simulink model "MPCtest1_real_44_180"  (Simulink 8.7)
settings: Solver=VariableStepAuto  StartTime=0.0  StopTime=16  RelTol=1e-3
libraries: neural x44, simulink x4, Solver_SF x1
(part 1 of 3)
settings Model: Creator=zch  LastModifiedBy=zch
settings DataIOCC: LimitDataPoints=off  SaveFormat=Dataset
settings DebuggingCC: UnderspecifiedInitializationDetection=Simplified  MergeDetectMultiDrivingBlocksExec=error
settings HardwareCC: ProdBitPerPointer=64  ProdLargestAtomicFloat=Float  ProdIntDivRoundTo=Zero  ProdEndianess=LittleEndian  ProdWordSize=64  ProdHWDeviceType=Intel->x86-64 (Windows64)
settings ModelReferenceCC: PropagateSignalLabelsOutOfModel=on
settings ConfigComp: CovModelRefEnable=off

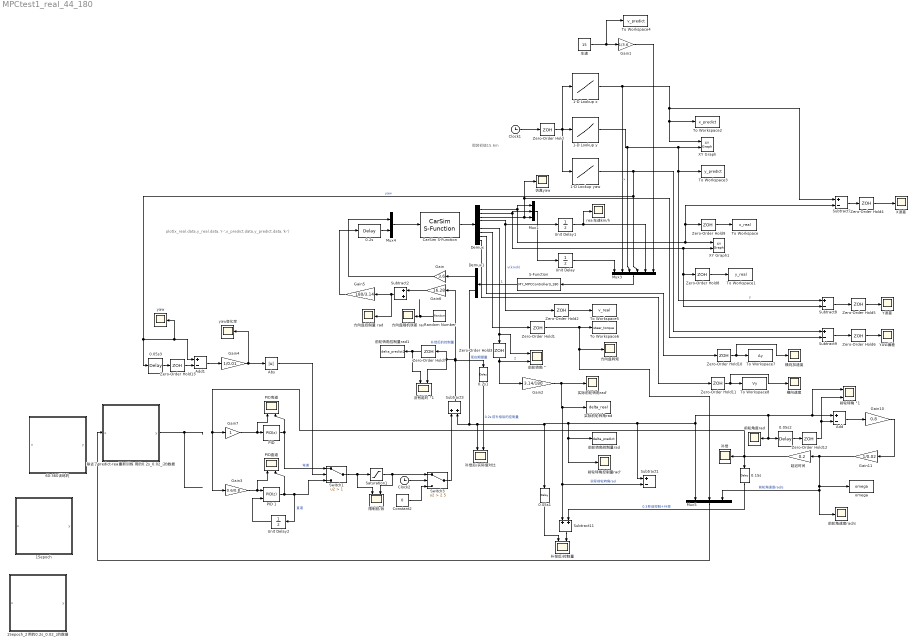
== system MPCtest1_real_44_180 ==
  note: plot(x_real.data,y_real.data,'r-',x_predict.data,y_predict.data,'k-')
  note: 假装初值15.6m
  0.05s1 : TransportDelay  DelayTime=0.05  PadeOrder=2
  0.05s2 : TransportDelay  DelayTime=0.02  PadeOrder=2
  0.05s3 : TransportDelay  DelayTime=0.01  PadeOrder=2
  0.15s : TransportDelay  DelayTime=0.15  PadeOrder=2
  0.2s : TransportDelay  DelayTime=0.2  PadeOrder=2
  0.2s1 : TransportDelay  DelayTime=0.2  PadeOrder=2
  1-D Lookup x : Lookup_n-D  NumberOfTableDimensions=1  BreakpointsForDimension1=|  Table=|  InternalRulePriority=Speed  RndMeth=Simplest  InputSameDT=on
      | [0
      | 0.018
      | 0.036
      | 0.054
      | 0.072
      | 0.09
      | 0.108
      | 0.126
      | 0.144
      | 0.162
      | 0.18
      | 0.198
      | 0.216
      | 0.234
      | 0.252
      | 0.27
      | 0.288
      | 0.306
      | 0.324
      | 0.342
      | 0.36
      | 0.378
      | 0.396
      | 0.414
      | 0.432
      | 0.45
      | 0.468
      | 0.486
      | 0.504
      | 0.522
      | 0.54
      | 0.558
      | 0.576
      | 0.594
      | 0.612
      | 0.63
      | 0.648
      | 0.666
      | 0.684
      | 0.702
      | 0.72
      | 0.738
      | 0.756
      | 0.774
      | 0.792
      | 0.81
      | 0.828
      | 0.846
      | 0.864
      | 0.882
      | 0.9
      | 0.918
      | 0.936
      | 0.954
      | 0.972
      | 0.99
      | 1.008
      | 1.026
      | 1.044
      | 1.062
      | 1.08
      | 1.098
      | 1.116
      | 1.134
      | 1.152
      | 1.17
      | 1.188
      | 1.206
      | 1.224
      | 1.242
      | 1.26
      | 1.278
      | 1.296
      | 1.314
      | 1.332
      | 1.35
      | 1.368
      | 1.386
      | 1.404
      | 1.422
      | 1.44
      | 1.458
      | 1.476
      | 1.494
      | 1.512
      | 1.53
      | 1.548
      | 1.566
      | 1.584
      | 1.602
      | 1.62
      | 1.638
      | 1.656
      | 1.674
      | 1.692
      | 1.71
      | 1.728
      | 1.746
      | 1.764
      | 1.782
      | 1.8
      | 1.818
      | 1.836
      | 1.854
      | 1.872
      | 1.89
      | 1.908
      | 1.926
      | 1.944
      | 1.962
      | 1.98
      | 1.998
      | 2.016
      | 2.034
      | 2.052
      | 2.07
      | 2.088
      | 2.106
      | 2.124
      | 2.142
      | 2.16
      | 2.178
      | 2.196
      | 2.214
      | 2.232
      | 2.25
      | 2.268
      | 2.286
      | 2.304
      | 2.322
      | 2.34
      | 2.358
      | 2.376
      | 2.394
      | 2.412
      | 2.43
      | 2.448
      | 2.466
      | 2.484
      | 2.502
      | 2.52
      | 2.538
      | 2.556
      | 2.574
      | 2.592
      | 2.61
      | 2.628
      | 2.646
      | 2.664
      | 2.682
      | 2.7
      | 2.718
      | 2.736
      | 2.754
      | 2.772
      | 2.79
      | 2.808
      | 2.826
      | 2.844
      | 2.862
      | 2.88
      | 2.898
      | 2.916
      | 2.934
      | 2.952
      | 2.97
      | 2.988
      | 3.006
      | 3.024
      | 3.042
      | 3.06
      | 3.078
      | 3.096
      | 3.114
      | 3.132
      | 3.15
      | 3.168
      | 3.186
      | 3.204
      | 3.222
      | 3.24
      | 3.258
      | 3.276
      | 3.294
      | 3.312
      | 3.33
      | 3.348
      | 3.366
      | 3.384
      | 3.402
      | 3.42
      | 3.438
      | 3.456
      | 3.474
      | 3.492
      | 3.51
      | 3.528
      | 3.546
      | 3.564
      | 3.582
      | 3.6
      | 3.61439994
      | 3.62879988
      | 3.64319982
      | 3.65759976
      | 3.6719997
      | 3.68639964
      | 3.70079958
      | 3.71519952
      | 3.72959946
      | 3.7439994
      | 3.75839934
      | 3.77279928
      | 3.78719922
      | 3.80159916
      | 3.8159991
      | 3.83039904
      | 3.84479898
      | 3.85919892
      | 3.87359886
      | 3.8879988
      | 3.90239874
      | 3.91679868
      | 3.93119862
      | 3.94559856
      | 3.9599985
      | 3.97439844
      | 3.98879838
      | 4.00319832
      | 4.01759826
      | 4.0319982
      | 4.04639814
      | 4.06079808
      | 4.07519802
      | 4.08959796
      | 4.1039979
      | 4.11839784
      | 4.13279778
      | 4.14719772
      | 4.16159766
      | 4.1759976
      | 4.19039754
      | 4.20479748
      | 4.21919742
      | 4.23359736
      | 4.2479973
      | 4.26239724
      | 4.27679718
      | 4.29119712
      | 4.30559706
      | 4.319997
      | 4.33439694
      | 4.34879688
      | 4.36319682
      | 4.37759676
      | 4.3919967
      | 4.40639664
      | 4.42079658
      | 4.43519652
      | 4.44959646
      | 4.4639964
      | 4.47839634
      | 4.49279628
      | 4.50719622
      | 4.52159616
      | 4.5359961
      | 4.55039604
      | 4.56479598
      | 4.57919592
      | 4.59359586
      | 4.6079958
      | 4.62239574
      | 4.63679568
      | 4.65119562
      | 4.66559556
      | 4.6799955
      | 4.69439544
      | 4.70879538
      | 4.72319532
      | 4.73759526
      | 4.7519952
      | 4.76639514
      | 4.78079508
      | 4.79519502
      | 4.80959496
      | 4.8239949
      | 4.83839484
      | 4.85279478
      | 4.86719472
      | 4.88159466
      | 4.8959946
      | 4.91039454
      | 4.92479448
      | 4.93919442
      | 4.95359436
      | 4.9679943
      | 4.98239424
      | 4.99679418
      | 5.01119412
      | 5.02559406
      | 5.039994
      | 5.05439394
      | 5.06879388
      | 5.08319382
      | 5.09759376
      | 5.1119937
      | 5.12639364
      | 5.14079358
      | 5.15519352
      | 5.16959346
      | 5.1839934
      | 5.19839334
      | 5.21279328
      | 5.22719322
      | 5.24159316
      | 5.2559931
      | 5.27039304
      | 5.28479298
      | 5.29919292
      | 5.31359286
      | 5.3279928
      | 5.34239274
      | 5.35679268
      | 5.37119262
      | 5.38559256
      | 5.3999925
      | 5.41439244
      | 5.42879238
      | 5.44319232
      | 5.45759226
      | 5.4719922
      | 5.48639214
      | 5.50079208
      | 5.51519202
      | 5.52959196
      | 5.5439919
      | 5.55839184
      | 5.57279178
      | 5.58719172
      | 5.60159166
      | 5.6159916
      | 5.63039154
      | 5.64479148
      | 5.65919142
      | 5.67359136
      | 5.6879913
      | 5.70239124
      | 5.71679118
      | 5.73119112
      | 5.74559106
      | 5.759991
      | 5.77439094
      | 5.78879088
      | 5.80319082
      | 5.81759076
      | 5.8319907
      | 5.84639064
      | 5.86079058
      | 5.87519052
      | 5.88959046
      | 5.9039904
      | 5.91839034
      | 5.93279028
      | 5.94719022
      | 5.96159016
      | 5.9759901
      | 5.99039004
      | 6.00478998
      | 6.01918992
      | 6.03358986
      | 6.0479898
      | 6.06238974
      | 6.07678968
      | 6.09118962
      | 6.10558956
      | 6.1199895
      | 6.13438944
      | 6.14878938
      | 6.16318932
      | 6.17758926
      | 6.1919892
      | 6.20638914
      | 6.22078908
      | 6.23518902
      | 6.24958896
      | 6.2639889
      | 6.27838884
      | 6.29278878
      | 6.30718872
      | 6.32158866
      | 6.3359886
      | 6.35038854
      | 6.36478848
      | 6.37918842
      | 6.39358836
      | 6.4079883
      | 6.42238824
      | 6.43678818
      | 6.45118812
      | 6.46558806
      | 6.479988
      | 6.49438794
      | 6.50878788
      | 6.52318782
      | 6.53758776
      | 6.5519877
      | 6.56638764
      | 6.58078758
      | 6.59518752
      | 6.60958746
      | 6.6239874
      | 6.63838734
      | 6.65278728
      | 6.66718722
      | 6.68158716
      | 6.6959871
      | 6.71038704
      | 6.72478698
      | 6.73918692
      | 6.75358686
      | 6.7679868
      | 6.78238674
      | 6.79678668
      | 6.81118662
      | 6.82558656
      | 6.8399865
      | 6.85438644
      | 6.86878638
      | 6.88318632
      | 6.89758626
      | 6.9119862
      | 6.92638614
      | 6.94078608
      | 6.95518602
      | 6.96958596
      | 6.9839859
      | 6.99838584
      | 7.01278578
      | 7.02718572
      | 7.04158566
      | 7.0559856
      | 7.07038554
      | 7.08478548
      | 7.09918542
      | 7.11358536
      | 7.1279853
      | 7.14238524
      | 7.15678518
      | 7.17118512
      | 7.18558506
      | 7.199985
      | 7.21438494
      | 7.22878488
      | 7.24318482
      | 7.25758476
      | 7.2719847
      | 7.28638464
      | 7.30078458
      | 7.31518452
      | 7.32958446
      | 7.3439844
      | 7.35838434
      | 7.37278428
      | 7.38718422
      | 7.40158416
      | 7.4159841
      | 7.43038404
      | 7.44478398
      | 7.45918392
      | 7.47358386
      | 7.4879838
      | 7.50238374
      | 7.51678368
      | 7.53118362
      | 7.54558356
      | 7.5599835
      | 7.57438344
      | 7.58878338
      | 7.60318332
      | 7.61758326
      | 7.6319832
      | 7.64638314
      | 7.66078308
      | 7.67518302
      | 7.68958296
      | 7.7039829
      | 7.71838284
      | 7.73278278
      | 7.74718272
      | 7.76158266
      | 7.7759826
      | 7.79038254
      | 7.80478248
      | 7.81918242
      | 7.83358236
      | 7.8479823
      | 7.86238224
      | 7.87678218
      | 7.89118212
      | 7.90558206
      | 7.919982
      | 7.93438194
      | 7.94878188
      | 7.96318182
      | 7.97758176
      | 7.9919817
      | 8.00638164
      | 8.02078158
      | 8.03518152
      | 8.04958146
      | 8.0639814
      | 8.07838134
      | 8.09278128
      | 8.10718122
      | 8.12158116
      | 8.123874581
      | 8.141874581
      | 8.159874581
      | 8.177874581
      | 8.195874581
      | 8.213874581
      | 8.231874581
      | 8.249874581
      | 8.267874581
      | 8.285874581
      | 8.303874581
      | 8.321874581
      | 8.339874581
      | 8.357874581
      | 8.375874581
      | 8.393874581
      | 8.411874581
      | 8.429874581
      | 8.447874581
      | 8.465874581
      | 8.483874581
      | 8.501874581
      | 8.519874581
      | 8.537874581
      | 8.555874581
      | 8.573874581
      | 8.591874581
      | 8.609874581
      | 8.627874581
      | 8.645874581
      | 8.663874581
      | 8.681874581
      | 8.699874581
      | 8.717874581
      | 8.735874581
      | 8.753874581
      | 8.771874581
      | 8.789874581
      | 8.807874581
      | 8.825874581
      | 8.843874581
      | 8.861874581
      | 8.879874581
      | 8.897874581
      | 8.915874581
      | 8.933874581
      | 8.951874581
      | 8.969874581
      | 8.987874581
      | 9.005874581
      | 9.023874581
      | 9.041874581
      | 9.059874581
      | 9.077874581
      | 9.095874581
      | 9.113874581
      | 9.131874581
      | 9.149874581
      | 9.167874581
      | 9.185874581
      | 9.203874581
      | 9.221874581
      | 9.239874581
      | 9.257874581
      | 9.275874581
      | 9.293874581
      | 9.311874581
      | 9.329874581
      | 9.347874581
      | 9.365874581
      | 9.383874581
      | 9.401874581
      | 9.419874581
      | 9.437874581
      | 9.455874581
      | 9.473874581
      | 9.491874581
      | 9.509874581
      | 9.527874581
      | 9.545874581
      | 9.563874581
      | 9.581874581
      | 9.599874581
      | 9.617874581
      | 9.635874581
      | 9.653874581
      | 9.671874581
      | 9.689874581
      | 9.707874581
      | 9.725874581
      | 9.743874581
      | 9.761874581
      | 9.779874581
      | 9.797874581
      | 9.815874581
      | 9.833874581
      | 9.851874581
      | 9.869874581
      | 9.887874581
      | 9.905874581
      | 9.923874581
      | 9.941874581
      | 9.959874581
      | 9.977874581
      | 9.995874581
      | 10.01387458
      | 10.03187458
      | 10.04987458
      | 10.06787458
      | 10.08587458
      | 10.10387458
      | 10.12187458
      | 10.13987458
      | 10.15787458
      | 10.17587458
      | 10.19387458
      | 10.21187458
      | 10.22987458
      | 10.24787458
      | 10.26587458
      | 10.28387458
      | 10.30187458
      | 10.31987458
      | 10.33787458
      | 10.35587458
      | 10.37387458
      | 10.39187458
      | 10.40987458
      | 10.42787458
      | 10.44587458
      | 10.46387458
      | 10.48187458
      | 10.49987458
      | 10.51787458
      | 10.53587458
      | 10.55387458
      | 10.57187458
      | 10.58987458
      | 10.60787458
      | 10.62587458
      | 10.64387458
      | 10.66187458
      | 10.67987458
      | 10.69787458
      | 10.71587458
      | 10.73387458
      | 10.75187458
      | 10.76987458
      | 10.78787458
      | 10.80587458
      | 10.82387458
      | 10.84187458
      | 10.85987458
      | 10.87787458
      | 10.89587458
      | 10.91387458
      | 10.93187458
      | 10.94987458
      | 10.96787458
      | 10.98587458
      | 11.00387458
      | 11.02187458
      | 11.03987458
      | 11.05787458
      | 11.07587458
      | 11.09387458
      | 11.11187458
      | 11.12987458
      | 11.14787458
      | 11.16587458
      | 11.18387458
      | 11.20187458
      | 11.21987458
      | 11.23787458
      | 11.25587458
      | 11.27387458
      | 11.29187458
      | 11.30987458
      | 11.32787458
      | 11.34587458
      | 11.36387458
      | 11.38187458
      | 11.39987458
      | 11.41787458
      | 11.43587458
      | 11.45387458
      | 11.47187458
      | 11.48987458
      | 11.50787458
      | 11.52587458
      | 11.54387458
      | 11.56187458
      | 11.57987458
      | 11.59787458
      | 11.61587458
      | 11.63387458
      | 11.65187458
      | 11.66987458
      | 11.68787458
      | 11.70587458
      | 11.72387458
      | ]*4/3
      | [0
      | 0.1
      | 0.2
      | 0.3
      | 0.4
      | 0.5
      | 0.6
      | 0.7
      | 0.8
      | 0.9
      | 1
      | 1.1
      | 1.2
      | 1.3
      | 1.4
      | 1.5
      | 1.6
      | 1.7
      | 1.8
      | 1.9
      | 2
      | 2.1
      | 2.2
      | 2.3
      | 2.4
      | 2.5
      | 2.6
      | 2.7
      | 2.8
      | 2.9
      | 3
      | 3.1
      | 3.2
      | 3.3
      | 3.4
      | 3.5
      | 3.6
      | 3.7
      | 3.8
      | 3.9
      | 4
      | 4.1
      | 4.2
      | 4.3
      | 4.4
      | 4.5
      | 4.6
      | 4.7
      | 4.8
      | 4.9
      | 5
      | 5.1
      | 5.2
      | 5.3
      | 5.4
      | 5.5
      | 5.6
      | 5.7
      | 5.8
      | 5.9
      | 6
      | 6.1
      | 6.2
      | 6.3
      | 6.4
      | 6.5
      | 6.6
      | 6.7
      | 6.8
      | 6.9
      | 7
      | 7.1
      | 7.2
      | 7.3
      | 7.4
      | 7.5
      | 7.6
      | 7.7
      | 7.8
      | 7.9
      | 8
      | 8.1
      | 8.2
      | 8.3
      | 8.4
      | 8.5
      | 8.6
      | 8.7
      | 8.8
      | 8.9
      | 9
      | 9.1
      | 9.2
      | 9.3
      | 9.4
      | 9.5
      | 9.6
      | 9.7
      | 9.8
      | 9.9
      | 10
      | 10.1
      | 10.2
      | 10.3
      | 10.4
      | 10.5
      | 10.6
      | 10.7
      | 10.8
      | 10.9
      | 11
      | 11.1
      | 11.2
      | 11.3
      | 11.4
      | 11.5
      | 11.6
      | 11.7
      | 11.8
      | 11.9
      | 12
      | 12.1
      | 12.2
      | 12.3
      | 12.4
      | 12.5
      | 12.6
      | 12.7
      | 12.8
      | 12.9
      | 13
      | 13.1
      | 13.2
      | 13.3
      | 13.4
      | 13.5
      | 13.6
      | 13.7
      | 13.8
      | 13.9
      | 14
      | 14.1
      | 14.2
      | 14.3
      | 14.4
      | 14.5
      | 14.6
      | 14.7
      | 14.8
      | 14.9
      | 15
      | 15.1
      | 15.2
      | 15.3
      | 15.4
      | 15.5
      | 15.6
      | 15.7
      | 15.8
      | 15.9
      | 16
      | 16.1
      | 16.2
      | 16.3
      | 16.4
      | 16.5
      | 16.6
      | 16.7
      | 16.8
      | 16.9
      | 17
      | 17.1
      | 17.2
      | 17.3
      | 17.4
      | 17.5
      | 17.6
      | 17.7
      | 17.8
      | 17.9
      | 18
      | 18.1
      | 18.2
      | 18.3
      | 18.4
      | 18.5
      | 18.6
      | 18.7
      | 18.8
      | 18.9
      | 19
      | 19.1
      | 19.2
      | 19.3
      | 19.4
      | 19.5
      | 19.6
      | 19.7
      | 19.8
      | 19.9
      | 20
      | 20.07999867
      | 20.15998933
      | 20.239964
      | 20.31991467
      | 20.39983335
      | 20.47971205
      | 20.55954278
      | 20.63931755
      | 20.71902839
      | 20.79866733
      | 20.87822641
      | 20.95769766
      | 21.03707314
      | 21.11634492
      | 21.19550506
      | 21.27454565
      | 21.35345879
      | 21.43223659
      | 21.51087116
      | 21.58935465
      | 21.6676792
      | 21.74583698
      | 21.82382019
      | 21.90162101
      | 21.97923167
      | 22.05664442
      | 22.13385149
      | 22.21084519
      | 22.2876178
      | 22.36416165
      | 22.44046909
      | 22.51653248
      | 22.59234423
      | 22.66789674
      | 22.74318246
      | 22.81819387
      | 22.89292346
      | 22.96736376
      | 23.04150732
      | 23.11534674
      | 23.18887462
      | 23.26208362
      | 23.33496642
      | 23.40751572
      | 23.47972427
      | 23.55158486
      | 23.62309028
      | 23.6942334
      | 23.76500711
      | 23.83540431
      | 23.90541798
      | 23.9750411
      | 24.04426673
      | 24.11308793
      | 24.18149783
      | 24.24948958
      | 24.31705639
      | 24.38419149
      | 24.45088818
      | 24.51713979
      | 24.58293968
      | 24.64828128
      | 24.71315806
      | 24.77756353
      | 24.84149125
      | 24.90493482
      | 24.9678879
      | 25.03034419
      | 25.09229746
      | 25.1537415
      | 25.21467017
      | 25.27507738
      | 25.33495708
      | 25.39430329
      | 25.45311008
      | 25.51137156
      | 25.56908191
      | 25.62623535
      | 25.68282618
      | 25.73884873
      | 25.79429739
      | 25.84916664
      | 25.90345097
      | 25.95714496
      | 26.01024324
      | 26.0627405
      | 26.1146315
      | 26.16591103
      | 26.21657398
      | 26.26661528
      | 26.31602992
      | 26.36481296
      | 26.41295953
      | 26.4604648
      | 26.50732404
      | 26.55353255
      | 26.59908571
      | 26.64397896
      | 26.68820783
      | 26.73176788
      | 26.77465476
      | 26.81686418
      | 26.85839191
      | 26.89923382
      | 26.9393858
      | 26.97884386
      | 27.01760403
      | 27.05566246
      | 27.09301532
      | 27.12965888
      | 27.16558949
      | 27.20080354
      | 27.23529752
      | 27.26906797
      | 27.30211152
      | 27.33442487
      | 27.36600478
      | 27.3968481
      | 27.42695174
      | 27.45631269
      | 27.48492801
      | 27.51279485
      | 27.53991042
      | 27.566272
      | 27.59187695
      | 27.61672273
      | 27.64080684
      | 27.66412688
      | 27.68668051
      | 27.70846548
      | 27.72947961
      | 27.7497208
      | 27.76918702
      | 27.78787633
      | 27.80578686
      | 27.82291682
      | 27.83926449
      | 27.85482824
      | 27.86960652
      | 27.88359784
      | 27.89680081
      | 27.9092141
      | 27.92083648
      | 27.93166679
      | 27.94170393
      | 27.95094691
      | 27.9593948
      | 27.96704676
      | 27.97390202
      | 27.97995989
      | 27.98521978
      | 27.98968115
      | 27.99334356
      | 27.99620664
      | 27.99827011
      | 27.99953376
      | 27.99999746
      | 27.99966117
      | 27.99852492
      | 27.99658882
      | 27.99385308
      | 27.99031795
      | 27.9859838
      | 27.98085105
      | 27.97492023
      | 27.96819192
      | 27.9606668
      | 27.95234562
      | 27.94322921
      | 27.93331848
      | 27.92261443
      | 27.91111813
      | 27.89883072
      | 27.88575343
      | 27.87188757
      | 27.85723454
      | 27.84179578
      | 27.82557285
      | 27.80856738
      | 27.79078105
      | 27.77221565
      | 27.75287303
      | 27.73275513
      | 27.71186397
      | 27.69020162
      | 27.66777026
      | 27.64457213
      | 27.62060955
      | 27.59588492
      | 27.5704007
      | 27.54415945
      | 27.51716379
      | 27.48941642
      | 27.46092011
      | 27.43167772
      | 27.40169217
      | 27.37096645
      | 27.33950364
      | 27.30730689
      | 27.27437941
      | 27.24072451
      | 27.20634553
      | 27.17124593
      | 27.13542921
      | 27.09889895
      | 27.06165881
      | 27.0237125
      | 26.98506384
      | 26.94571667
      | 26.90567493
      | 26.86494264
      | 26.82352385
      | 26.78142272
      | 26.73864345
      | 26.69519033
      | 26.65106769
      | 26.60627994
      | 26.56083158
      | 26.51472714
      | 26.46797123
      | 26.42056853
      | 26.37252378
      | 26.32384178
      | 26.2745274
      | 26.22458558
      | 26.1740213
      | 26.12283962
      | 26.07104567
      | 26.01864461
      | 25.9656417
      | 25.91204222
      | 25.85785155
      | 25.8030751
      | 25.74771834
      | 25.69178682
      | 25.63528613
      | 25.57822191
      | 25.52059987
      | 25.46242578
      | 25.40370544
      | 25.34444475
      | 25.28464961
      | 25.22432601
      | 25.16347999
      | 25.10211762
      | 25.04024504
      | 24.97786844
      | 24.91499406
      | 24.85162819
      | 24.78777715
      | 24.72344734
      | 24.6586452
      | 24.59337719
      | 24.52764984
      | 24.46146974
      | 24.39484349
      | 24.32777776
      | 24.26027926
      | 24.19235473
      | 24.12401097
      | 24.05525482
      | 23.98609314
      | 23.91653285
      | 23.84658092
      | 23.77624433
      | 23.70553012
      | 23.63444536
      | 23.56299716
      | 23.49119266
      | 23.41903904
      | 23.34654353
      | 23.27371336
      | 23.20055582
      | 23.12707823
      | 23.05328794
      | 22.97919232
      | 22.90479878
      | 22.83011476
      | 22.75514774
      | 22.6799052
      | 22.60439468
      | 22.52862371
      | 22.45259989
      | 22.37633081
      | 22.2998241
      | 22.22308741
      | 22.14612841
      | 22.0689548
      | 21.99157429
      | 21.91399463
      | 21.83622358
      | 21.7582689
      | 21.68013839
      | 21.60183988
      | 21.52338118
      | 21.44477014
      | 21.36601463
      | 21.28712252
      | 21.2081017
      | 21.12896006
      | 21.04970554
      | 20.97034604
      | 20.89088951
      | 20.81134389
      | 20.73171714
      | 20.65201721
      | 20.57225209
      | 20.49242974
      | 20.41255815
      | 20.3326453
      | 20.25269919
      | 20.17272781
      | 20.09273915
      | 20.01274122
      | 20
      | 19.9
      | 19.8
      | 19.7
      | 19.6
      | 19.5
      | 19.4
      | 19.3
      | 19.2
      | 19.1
      | 19
      | 18.9
      | 18.8
      | 18.7
      | 18.6
      | 18.5
      | 18.4
      | 18.3
      | 18.2
      | 18.1
      | 18
      | 17.9
      | 17.8
      | 17.7
      | 17.6
      | 17.5
      | 17.4
      | 17.3
      | 17.2
      | 17.1
      | 17
      | 16.9
      | 16.8
      | 16.7
      | 16.6
      | 16.5
      | 16.4
      | 16.3
      | 16.2
      | 16.1
      | 16
      | 15.9
      | 15.8
      | 15.7
      | 15.6
      | 15.5
      | 15.4
      | 15.3
      | 15.2
      | 15.1
      | 15
      | 14.9
      | 14.8
      | 14.7
      | 14.6
      | 14.5
      | 14.4
      | 14.3
      | 14.2
      | 14.1
      | 14
      | 13.9
      | 13.8
      | 13.7
      | 13.6
      | 13.5
      | 13.4
      | 13.3
      | 13.2
      | 13.1
      | 13
      | 12.9
      | 12.8
      | 12.7
      | 12.6
      | 12.5
      | 12.4
      | 12.3
      | 12.2
      | 12.1
      | 12
      | 11.9
      | 11.8
      | 11.7
      | 11.6
      | 11.5
      | 11.4
      | 11.3
      | 11.2
      | 11.1
      | 11
      | 10.9
      | 10.8
      | 10.7
      | 10.6
      | 10.5
      | 10.4
      | 10.3
      | 10.2
      | 10.1
      | 10
      | 9.9
      | 9.8
      | 9.7
      | 9.6
      | 9.5
      | 9.4
      | 9.3
      | 9.2
      | 9.1
      | 9
      | 8.9
      | 8.8
      | 8.7
      | 8.6
      | 8.5
      | 8.4
      | 8.3
      | 8.2
      | 8.1
      | 8
      | 7.9
      | 7.8
      | 7.7
      | 7.6
      | 7.5
      | 7.4
      | 7.3
      | 7.2
      | 7.1
      | 7
      | 6.9
      | 6.8
      | 6.7
      | 6.6
      | 6.5
      | 6.4
      | 6.3
      | 6.2
      | 6.1
      | 6
      | 5.9
      | 5.8
      | 5.7
      | 5.6
      | 5.5
      | 5.4
      | 5.3
      | 5.2
      | 5.1
      | 5
      | 4.9
      | 4.8
      | 4.7
      | 4.6
      | 4.5
      | 4.4
      | 4.3
      | 4.2
      | 4.1
      | 4
      | 3.9
      | 3.8
      | 3.7
      | 3.6
      | 3.5
      | 3.4
      | 3.3
      | 3.2
      | 3.1
      | 3
      | 2.9
      | 2.8
      | 2.7
      | 2.6
      | 2.5
      | 2.4
      | 2.3
      | 2.2
      | 2.1
      | 2
      | 1.9
      | 1.8
      | 1.7
      | 1.6
      | 1.5
      | 1.4
      | 1.3
      | 1.2
      | 1.1
      | 1
      | 0.9
      | 0.8
      | 0.7
      | 0.6
      | 0.5
      | 0.4
      | 0.3
      | 0.2
      | 0.1
      | 0
      | ]
  1-D Lookup y : Lookup_n-D  NumberOfTableDimensions=1  BreakpointsForDimension1=|  Table=|  InternalRulePriority=Speed  RndMeth=Simplest  InputSameDT=on
      | [0
      | 0.018
      | 0.036
      | 0.054
      | 0.072
      | 0.09
      | 0.108
      | 0.126
      | 0.144
      | 0.162
      | 0.18
      | 0.198
      | 0.216
      | 0.234
      | 0.252
      | 0.27
      | 0.288
      | 0.306
      | 0.324
      | 0.342
      | 0.36
      | 0.378
      | 0.396
      | 0.414
      | 0.432
      | 0.45
      | 0.468
      | 0.486
      | 0.504
      | 0.522
      | 0.54
      | 0.558
      | 0.576
      | 0.594
      | 0.612
      | 0.63
      | 0.648
      | 0.666
      | 0.684
      | 0.702
      | 0.72
      | 0.738
      | 0.756
      | 0.774
      | 0.792
      | 0.81
      | 0.828
      | 0.846
      | 0.864
      | 0.882
      | 0.9
      | 0.918
      | 0.936
      | 0.954
      | 0.972
      | 0.99
      | 1.008
      | 1.026
      | 1.044
      | 1.062
      | 1.08
      | 1.098
      | 1.116
      | 1.134
      | 1.152
      | 1.17
      | 1.188
      | 1.206
      | 1.224
      | 1.242
      | 1.26
      | 1.278
      | 1.296
      | 1.314
      | 1.332
      | 1.35
      | 1.368
      | 1.386
      | 1.404
      | 1.422
      | 1.44
      | 1.458
      | 1.476
      | 1.494
      | 1.512
      | 1.53
      | 1.548
      | 1.566
      | 1.584
      | 1.602
      | 1.62
      | 1.638
      | 1.656
      | 1.674
      | 1.692
      | 1.71
      | 1.728
      | 1.746
      | 1.764
      | 1.782
      | 1.8
      | 1.818
      | 1.836
      | 1.854
      | 1.872
      | 1.89
      | 1.908
      | 1.926
      | 1.944
      | 1.962
      | 1.98
      | 1.998
      | 2.016
      | 2.034
      | 2.052
      | 2.07
      | 2.088
      | 2.106
      | 2.124
      | 2.142
      | 2.16
      | 2.178
      | 2.196
      | 2.214
      | 2.232
      | 2.25
      | 2.268
      | 2.286
      | 2.304
      | 2.322
      | 2.34
      | 2.358
      | 2.376
      | 2.394
      | 2.412
      | 2.43
      | 2.448
      | 2.466
      | 2.484
      | 2.502
      | 2.52
      | 2.538
      | 2.556
      | 2.574
      | 2.592
      | 2.61
      | 2.628
      | 2.646
      | 2.664
      | 2.682
      | 2.7
      | 2.718
      | 2.736
      | 2.754
      | 2.772
      | 2.79
      | 2.808
      | 2.826
      | 2.844
      | 2.862
      | 2.88
      | 2.898
      | 2.916
      | 2.934
      | 2.952
      | 2.97
      | 2.988
      | 3.006
      | 3.024
      | 3.042
      | 3.06
      | 3.078
      | 3.096
      | 3.114
      | 3.132
      | 3.15
      | 3.168
      | 3.186
      | 3.204
      | 3.222
      | 3.24
      | 3.258
      | 3.276
      | 3.294
      | 3.312
      | 3.33
      | 3.348
      | 3.366
      | 3.384
      | 3.402
      | 3.42
      | 3.438
      | 3.456
      | 3.474
      | 3.492
      | 3.51
      | 3.528
      | 3.546
      | 3.564
      | 3.582
      | 3.6
      | 3.61439994
      | 3.62879988
      | 3.64319982
      | 3.65759976
      | 3.6719997
      | 3.68639964
      | 3.70079958
      | 3.71519952
      | 3.72959946
      | 3.7439994
      | 3.75839934
      | 3.77279928
      | 3.78719922
      | 3.80159916
      | 3.8159991
      | 3.83039904
      | 3.84479898
      | 3.85919892
      | 3.87359886
      | 3.8879988
      | 3.90239874
      | 3.91679868
      | 3.93119862
      | 3.94559856
      | 3.9599985
      | 3.97439844
      | 3.98879838
      | 4.00319832
      | 4.01759826
      | 4.0319982
      | 4.04639814
      | 4.06079808
      | 4.07519802
      | 4.08959796
      | 4.1039979
      | 4.11839784
      | 4.13279778
      | 4.14719772
      | 4.16159766
      | 4.1759976
      | 4.19039754
      | 4.20479748
      | 4.21919742
      | 4.23359736
      | 4.2479973
      | 4.26239724
      | 4.27679718
      | 4.29119712
      | 4.30559706
      | 4.319997
      | 4.33439694
      | 4.34879688
      | 4.36319682
      | 4.37759676
      | 4.3919967
      | 4.40639664
      | 4.42079658
      | 4.43519652
      | 4.44959646
      | 4.4639964
      | 4.47839634
      | 4.49279628
      | 4.50719622
      | 4.52159616
      | 4.5359961
      | 4.55039604
      | 4.56479598
      | 4.57919592
      | 4.59359586
      | 4.6079958
      | 4.62239574
      | 4.63679568
      | 4.65119562
      | 4.66559556
      | 4.6799955
      | 4.69439544
      | 4.70879538
      | 4.72319532
      | 4.73759526
      | 4.7519952
      | 4.76639514
      | 4.78079508
      | 4.79519502
      | 4.80959496
      | 4.8239949
      | 4.83839484
      | 4.85279478
      | 4.86719472
      | 4.88159466
      | 4.8959946
      | 4.91039454
      | 4.92479448
      | 4.93919442
      | 4.95359436
      | 4.9679943
      | 4.98239424
      | 4.99679418
      | 5.01119412
      | 5.02559406
      | 5.039994
      | 5.05439394
      | 5.06879388
      | 5.08319382
      | 5.09759376
      | 5.1119937
      | 5.12639364
      | 5.14079358
      | 5.15519352
      | 5.16959346
      | 5.1839934
      | 5.19839334
      | 5.21279328
      | 5.22719322
      | 5.24159316
      | 5.2559931
      | 5.27039304
      | 5.28479298
      | 5.29919292
      | 5.31359286
      | 5.3279928
      | 5.34239274
      | 5.35679268
      | 5.37119262
      | 5.38559256
      | 5.3999925
      | 5.41439244
      | 5.42879238
      | 5.44319232
      | 5.45759226
      | 5.4719922
      | 5.48639214
      | 5.50079208
      | 5.51519202
      | 5.52959196
      | 5.5439919
      | 5.55839184
      | 5.57279178
      | 5.58719172
      | 5.60159166
      | 5.6159916
      | 5.63039154
      | 5.64479148
      | 5.65919142
      | 5.67359136
      | 5.6879913
      | 5.70239124
      | 5.71679118
      | 5.73119112
      | 5.74559106
      | 5.759991
      | 5.77439094
      | 5.78879088
      | 5.80319082
      | 5.81759076
      | 5.8319907
      | 5.84639064
      | 5.86079058
      | 5.87519052
      | 5.88959046
      | 5.9039904
      | 5.91839034
      | 5.93279028
      | 5.94719022
      | 5.96159016
      | 5.9759901
      | 5.99039004
      | 6.00478998
      | 6.01918992
      | 6.03358986
      | 6.0479898
      | 6.06238974
      | 6.07678968
      | 6.09118962
      | 6.10558956
      | 6.1199895
      | 6.13438944
      | 6.14878938
      | 6.16318932
      | 6.17758926
      | 6.1919892
      | 6.20638914
      | 6.22078908
      | 6.23518902
      | 6.24958896
      | 6.2639889
      | 6.27838884
      | 6.29278878
      | 6.30718872
      | 6.32158866
      | 6.3359886
      | 6.35038854
      | 6.36478848
      | 6.37918842
      | 6.39358836
      | 6.4079883
      | 6.42238824
      | 6.43678818
      | 6.45118812
      | 6.46558806
      | 6.479988
      | 6.49438794
      | 6.50878788
      | 6.52318782
      | 6.53758776
      | 6.5519877
      | 6.56638764
      | 6.58078758
      | 6.59518752
      | 6.60958746
      | 6.6239874
      | 6.63838734
      | 6.65278728
      | 6.66718722
      | 6.68158716
      | 6.6959871
      | 6.71038704
      | 6.72478698
      | 6.73918692
      | 6.75358686
      | 6.7679868
      | 6.78238674
      | 6.79678668
      | 6.81118662
      | 6.82558656
      | 6.8399865
      | 6.85438644
      | 6.86878638
      | 6.88318632
      | 6.89758626
      | 6.9119862
      | 6.92638614
      | 6.94078608
      | 6.95518602
      | 6.96958596
      | 6.9839859
      | 6.99838584
      | 7.01278578
      | 7.02718572
      | 7.04158566
      | 7.0559856
      | 7.07038554
      | 7.08478548
      | 7.09918542
      | 7.11358536
      | 7.1279853
      | 7.14238524
      | 7.15678518
      | 7.17118512
      | 7.18558506
      | 7.199985
      | 7.21438494
      | 7.22878488
      | 7.24318482
      | 7.25758476
      | 7.2719847
      | 7.28638464
      | 7.30078458
      | 7.31518452
      | 7.32958446
      | 7.3439844
      | 7.35838434
      | 7.37278428
      | 7.38718422
      | 7.40158416
      | 7.4159841
      | 7.43038404
      | 7.44478398
      | 7.45918392
      | 7.47358386
      | 7.4879838
      | 7.50238374
      | 7.51678368
      | 7.53118362
      | 7.54558356
      | 7.5599835
      | 7.57438344
      | 7.58878338
      | 7.60318332
      | 7.61758326
      | 7.6319832
      | 7.64638314
      | 7.66078308
      | 7.67518302
      | 7.68958296
      | 7.7039829
      | 7.71838284
      | 7.73278278
      | 7.74718272
      | 7.76158266
      | 7.7759826
      | 7.79038254
      | 7.80478248
      | 7.81918242
      | 7.83358236
      | 7.8479823
      | 7.86238224
      | 7.87678218
      | 7.89118212
      | 7.90558206
      | 7.919982
      | 7.93438194
      | 7.94878188
      | 7.96318182
      | 7.97758176
      | 7.9919817
      | 8.00638164
      | 8.02078158
      | 8.03518152
      | 8.04958146
      | 8.0639814
      | 8.07838134
      | 8.09278128
      | 8.10718122
      | 8.12158116
      | 8.123874581
      | 8.141874581
      | 8.159874581
      | 8.177874581
      | 8.195874581
      | 8.213874581
      | 8.231874581
      | 8.249874581
      | 8.267874581
      | 8.285874581
      | 8.303874581
      | 8.321874581
      | 8.339874581
      | 8.357874581
      | 8.375874581
      | 8.393874581
      | 8.411874581
      | 8.429874581
      | 8.447874581
      | 8.465874581
      | 8.483874581
      | 8.501874581
      | 8.519874581
      | 8.537874581
      | 8.555874581
      | 8.573874581
      | 8.591874581
      | 8.609874581
      | 8.627874581
      | 8.645874581
      | 8.663874581
      | 8.681874581
      | 8.699874581
      | 8.717874581
      | 8.735874581
      | 8.753874581
      | 8.771874581
      | 8.789874581
      | 8.807874581
      | 8.825874581
      | 8.843874581
      | 8.861874581
      | 8.879874581
      | 8.897874581
      | 8.915874581
      | 8.933874581
      | 8.951874581
      | 8.969874581
      | 8.987874581
      | 9.005874581
      | 9.023874581
      | 9.041874581
      | 9.059874581
      | 9.077874581
      | 9.095874581
      | 9.113874581
      | 9.131874581
      | 9.149874581
      | 9.167874581
      | 9.185874581
      | 9.203874581
      | 9.221874581
      | 9.239874581
      | 9.257874581
      | 9.275874581
      | 9.293874581
      | 9.311874581
      | 9.329874581
      | 9.347874581
      | 9.365874581
      | 9.383874581
      | 9.401874581
      | 9.419874581
      | 9.437874581
      | 9.455874581
      | 9.473874581
      | 9.491874581
      | 9.509874581
      | 9.527874581
      | 9.545874581
      | 9.563874581
      | 9.581874581
      | 9.599874581
      | 9.617874581
      | 9.635874581
      | 9.653874581
      | 9.671874581
      | 9.689874581
      | 9.707874581
      | 9.725874581
      | 9.743874581
      | 9.761874581
      | 9.779874581
      | 9.797874581
      | 9.815874581
      | 9.833874581
      | 9.851874581
      | 9.869874581
      | 9.887874581
      | 9.905874581
      | 9.923874581
      | 9.941874581
      | 9.959874581
      | 9.977874581
      | 9.995874581
      | 10.01387458
      | 10.03187458
      | 10.04987458
      | 10.06787458
      | 10.08587458
      | 10.10387458
      | 10.12187458
      | 10.13987458
      | 10.15787458
      | 10.17587458
      | 10.19387458
      | 10.21187458
      | 10.22987458
      | 10.24787458
      | 10.26587458
      | 10.28387458
      | 10.30187458
      | 10.31987458
      | 10.33787458
      | 10.35587458
      | 10.37387458
      | 10.39187458
      | 10.40987458
      | 10.42787458
      | 10.44587458
      | 10.46387458
      | 10.48187458
      | 10.49987458
      | 10.51787458
      | 10.53587458
      | 10.55387458
      | 10.57187458
      | 10.58987458
      | 10.60787458
      | 10.62587458
      | 10.64387458
      | 10.66187458
      | 10.67987458
      | 10.69787458
      | 10.71587458
      | 10.73387458
      | 10.75187458
      | 10.76987458
      | 10.78787458
      | 10.80587458
      | 10.82387458
      | 10.84187458
      | 10.85987458
      | 10.87787458
      | 10.89587458
      | 10.91387458
      | 10.93187458
      | 10.94987458
      | 10.96787458
      | 10.98587458
      | 11.00387458
      | 11.02187458
      | 11.03987458
      | 11.05787458
      | 11.07587458
      | 11.09387458
      | 11.11187458
      | 11.12987458
      | 11.14787458
      | 11.16587458
      | 11.18387458
      | 11.20187458
      | 11.21987458
      | 11.23787458
      | 11.25587458
      | 11.27387458
      | 11.29187458
      | 11.30987458
      | 11.32787458
      | 11.34587458
      | 11.36387458
      | 11.38187458
      | 11.39987458
      | 11.41787458
      | 11.43587458
      | 11.45387458
      | 11.47187458
      | 11.48987458
      | 11.50787458
      | 11.52587458
      | 11.54387458
      | 11.56187458
      | 11.57987458
      | 11.59787458
      | 11.61587458
      | 11.63387458
      | 11.65187458
      | 11.66987458
      | 11.68787458
      | 11.70587458
      | 11.72387458
      | ]*4/3
      | [0
      | 0
      | 0
      | 0
      | 0
      | 0
      | 0
      | 0
      | 0
      | 0
      | 0
      | 0
      | 0
      | 0
      | 0
      | 0
      | 0
      | 0
      | 0
      | 0
      | 0
      | 0
      | 0
      | 0
      | 0
      | 0
      | 0
      | 0
      | 0
      | 0
      | 0
      | 0
      | 0
      | 0
      | 0
      | 0
      | 0
      | 0
      | 0
      | 0
      | 0
      | 0
      | 0
      | 0
      | 0
      | 0
      | 0
      | 0
      | 0
      | 0
      | 0
      | 0
      | 0
      | 0
      | 0
      | 0
      | 0
      | 0
      | 0
      | 0
      | 0
      | 0
      | 0
      | 0
      | 0
      | 0
      | 0
      | 0
      | 0
      | 0
      | 0
      | 0
      | 0
      | 0
      | 0
      | 0
      | 0
      | 0
      | 0
      | 0
      | 0
      | 0
      | 0
      | 0
      | 0
      | 0
      | 0
      | 0
      | 0
      | 0
      | 0
      | 0
      | 0
      | 0
      | 0
      | 0
      | 0
      | 0
      | 0
      | 0
      | 0
      | 0
      | 0
      | 0
      | 0
      | 0
      | 0
      | 0
      | 0
      | 0
      | 0
      | 0
      | 0
      | 0
      | 0
      | 0
      | 0
      | 0
      | 0
      | 0
      | 0
      | 0
      | 0
      | 0
      | 0
      | 0
      | 0
      | 0
      | 0
      | 0
      | 0
      | 0
      | 0
      | 0
      | 0
      | 0
      | 0
      | 0
      | 0
      | 0
      | 0
      | 0
      | 0
      | 0
      | 0
      | 0
      | 0
      | 0
      | 0
      | 0
      | 0
      | 0.00E+00
      | 0.00E+00
      | 0.00E+00
      | 0.00E+00
      | 0.00E+00
      | 0
      | 0
      | 0
      | 0
      | 0
      | 0
      | 0
      | 0
      | 0
      | 0
      | 0
      | 0
      | 0
      | 0
      | 0
      | 0
      | 0
      | 0
      | 0
      | 0
      | 0
      | 0
      | 0
      | 0
      | 0
      | 0
      | 0
      | 0
      | 0
      | 0
      | 0
      | 0
      | 0
      | 0
      | 0
      | 0
      | 0
      | 0
      | 0
      | 0
      | 0
      | 0
      | 0
      | 0
      | 0
      | 0.000399997
      | 0.001599947
      | 0.00359973
      | 0.006399147
      | 0.009997917
      | 0.014395681
      | 0.019591998
      | 0.02558635
      | 0.032378136
      | 0.039966678
      | 0.048351216
      | 0.057530913
      | 0.06750485
      | 0.07827203
      | 0.089831377
      | 0.102181733
      | 0.115321865
      | 0.129250458
      | 0.143966119
      | 0.159467377
      | 0.175752682
      | 0.192820405
      | 0.21066884
      | 0.229296201
      | 0.248700626
      | 0.268880175
      | 0.289832829
      | 0.311556494
      | 0.334048996
      | 0.357308087
      | 0.381331441
      | 0.406116655
      | 0.431661252
      | 0.457962676
      | 0.485018297
      | 0.512825411
      | 0.541381235
      | 0.570682915
      | 0.600727521
      | 0.631512048
      | 0.663033417
      | 0.695288478
      | 0.728274003
      | 0.761986694
      | 0.796423181
      | 0.83158002
      | 0.867453694
      | 0.904040618
      | 0.941337131
      | 0.979339505
      | 1.018043939
      | 1.057446563
      | 1.097543436
      | 1.138330549
      | 1.179803824
      | 1.221959112
      | 1.264792199
      | 1.308298801
      | 1.352474567
      | 1.397315081
      | 1.442815857
      | 1.488972347
      | 1.535779934
      | 1.583233937
      | 1.631329612
      | 1.680062148
      | 1.729426673
      | 1.77941825
      | 1.83003188
      | 1.881262502
      | 1.933104992
      | 1.985554167
      | 2.038604781
      | 2.09225153
      | 2.146489049
      | 2.201311914
      | 2.256714643
      | 2.312691696
      | 2.369237475
      | 2.426346325
      | 2.484012536
      | 2.542230342
      | 2.600993919
      | 2.660297393
      | 2.720134833
      | 2.780500255
      | 2.841387622
      | 2.902790846
      | 2.964703787
      | 3.027120254
      | 3.090034004
      | 3.153438747
      | 3.217328142
      | 3.2816958
      | 3.346535284
      | 3.411840111
      | 3.477603751
      | 3.543819626
      | 3.610481115
      | 3.677581553
      | 3.745114229
      | 3.81307239
      | 3.88144924
      | 3.950237942
      | 4.019431617
      | 4.089023345
      | 4.159006168
      | 4.229373087
      | 4.300117065
      | 4.371231029
      | 4.442707866
      | 4.51454043
      | 4.586721537
      | 4.659243968
      | 4.732100473
      | 4.805283765
      | 4.878786526
      | 4.952601405
      | 5.026721022
      | 5.101137964
      | 5.17584479
      | 5.250834029
      | 5.326098183
      | 5.401629724
      | 5.477421101
      | 5.553464733
      | 5.629753017
      | 5.706278323
      | 5.783033
      | 5.860009371
      | 5.93719974
      | 6.014596387
      | 6.092191573
      | 6.169977538
      | 6.247946503
      | 6.326090673
      | 6.404402232
      | 6.48287335
      | 6.561496179
      | 6.640262857
      | 6.719165508
      | 6.798196241
      | 6.877347153
      | 6.95661033
      | 7.035977845
      | 7.115441761
      | 7.194994133
      | 7.274627004
      | 7.354332412
      | 7.434102387
      | 7.51392895
      | 7.593804121
      | 7.67371991
      | 7.753668327
      | 7.833641378
      | 7.913631064
      | 7.993629386
      | 8.073628346
      | 8.153619943
      | 8.233596178
      | 8.313549054
      | 8.393470575
      | 8.47335275
      | 8.553187589
      | 8.63296711
      | 8.712683335
      | 8.792328293
      | 8.871894018
      | 8.951372554
      | 9.030755954
      | 9.11003628
      | 9.189205602
      | 9.268256005
      | 9.347179584
      | 9.425968445
      | 9.504614711
      | 9.583110517
      | 9.661448013
      | 9.739619365
      | 9.817616758
      | 9.895432389
      | 9.97305848
      | 10.05048727
      | 10.127711
      | 10.20472197
      | 10.28151247
      | 10.35807482
      | 10.43440137
      | 10.51048447
      | 10.58631653
      | 10.66188997
      | 10.73719721
      | 10.81223074
      | 10.88698304
      | 10.96144665
      | 11.03561412
      | 11.10947803
      | 11.18303099
      | 11.25626565
      | 11.32917469
      | 11.40175082
      | 11.47398677
      | 11.54587533
      | 11.6174093
      | 11.68858153
      | 11.75938491
      | 11.82981235
      | 11.89985682
      | 11.9695113
      | 12.03876884
      | 12.1076225
      | 12.1760654
      | 12.2440907
      | 12.3116916
      | 12.37886132
      | 12.44559317
      | 12.51188046
      | 12.57771657
      | 12.64309491
      | 12.70800894
      | 12.77245217
      | 12.83641817
      | 12.89990053
      | 12.9628929
      | 13.02538898
      | 13.08738253
      | 13.14886735
      | 13.20983728
      | 13.27028624
      | 13.33020817
      | 13.38959708
      | 13.44844704
      | 13.50675216
      | 13.56450661
      | 13.62170461
      | 13.67834045
      | 13.73440846
      | 13.78990303
      | 13.84481862
      | 13.89914972
      | 13.95289092
      | 14.00603684
      | 14.05858215
      | 14.11052162
      | 14.16185003
      | 14.21256227
      | 14.26265325
      | 14.31211798
      | 14.3609515
      | 14.40914892
      | 14.45670544
      | 14.5036163
      | 14.54987679
      | 14.59548231
      | 14.64042828
      | 14.68471022
      | 14.72832369
      | 14.77126433
      | 14.81352785
      | 14.85511003
      | 14.8960067
      | 14.93621377
      | 14.97572723
      | 15.01454312
      | 15.05265757
      | 15.09006675
      | 15.12676693
      | 15.16275445
      | 15.19802569
      | 15.23257714
      | 15.26640533
      | 15.29950689
      | 15.33187851
      | 15.36351694
      | 15.39441903
      | 15.42458168
      | 15.45400188
      | 15.48267669
      | 15.51060323
      | 15.53777873
      | 15.56420044
      | 15.58986575
      | 15.61477208
      | 15.63891693
      | 15.6622979
      | 15.68491265
      | 15.70675891
      | 15.7278345
      | 15.74813731
      | 15.76766532
      | 15.78641657
      | 15.80438918
      | 15.82158136
      | 15.83799139
      | 15.85361762
      | 15.8684585
      | 15.88251255
      | 15.89577834
      | 15.90825457
      | 15.91993997
      | 15.93083339
      | 15.94093373
      | 15.95023999
      | 15.95875123
      | 15.9664666
      | 15.97338533
      | 15.97950672
      | 15.98483018
      | 15.98935515
      | 15.9930812
      | 15.99600795
      | 15.9981351
      | 15.99946245
      | 15.99998985
      | 16
      | 16
      | 16
      | 16
      | 16
      | 16
      | 16
      | 16
      | 16
      | 16
      | 16
      | 16
      | 16
      | 16
      | 16
      | 16
      | 16
      | 16
      | 16
      | 16
      | 16
      | 16
      | 16
      | 16
      | 16
      | 16
      | 16
      | 16
      | 16
      | 16
      | 16
      | 16
      | 16
      | 16
      | 16
      | 16
      | 1.60E+01
      | 1.60E+01
      | 16
      | 16
      | 16
      | 16
      | 16
      | 16
      | 16
      | 16
      | 16
      | 16
      | 16
      | 16
      | 16
      | 16
      | 16
      | 16
      | 16
      | 16
      | 16
      | 16
      | 16
      | 16
      | 16
      | 16
      | 16
      | 16
      | 16
      | 16
      | 16
      | 16
      | 16
      | 16
      | 16
      | 16
      | 16
      | 16
      | 16
      | 16
      | 16
      | 16
      | 16
      | 16
      | 16
      | 16
      | 16
      | 16
      | 16
      | 16
      | 16
      | 16
      | 16
      | 1.60E+01
      | 1.60E+01
      | 1.60E+01
      | 1.60E+01
      | 1.60E+01
      | 1.60E+01
      | 16
      | 1.60E+01
      | 1.60E+01
      | 1.60E+01
      | 1.60E+01
      | 1.60E+01
      | 1.60E+01
      | 1.60E+01
      | 16
      | 16
      | 16
      | 16
      | 16
      | 16
      | 16
      | 16
      | 16
      | 16
      | 16
      | 16
      | 16
      | 16
      | 16
      | 16
      | 16
      | 16
      | 16
      | 16
      | 16
      | 16
      | 16
      | 16
      | 16
      | 16
      | 16
      | 16
      | 1.60E+01
      | 1.60E+01
      | 1.60E+01
      | 1.60E+01
      | 16
      | 1.60E+01
      | 1.60E+01
      | 16
      | 16
      | 16
      | 16
      | 16
      | 16
      | 16
      | 16
      | 16
      | 16
      | 16
      | 16
      | 16
      | 16
      | 16
      | 16
      | 16
      | 16
      | 16
      | 16
      | 16
      | 16
      | 16
      | 16
      | 16
      | 16
      | 16
      | 16
      | 16
      | 16
      | 16
      | 16
      | 16
      | 16
      | 16
      | 16
      | 16
      | 16
      | 16
      | 16
      | 16
      | 16
      | 16
      | 16
      | 16
      | 16
      | 16
      | 16
      | 16
      | 16
      | 16
      | 16
      | 16
      | 16
      | 16
      | 16
      | 16
      | 16
      | 16
      | 16
      | 16
      | 16
      | 16
      | ]
  1-D Lookup yaw : Lookup_n-D  NumberOfTableDimensions=1  BreakpointsForDimension1=|  Table=|  InternalRulePriority=Speed  RndMeth=Simplest  InputSameDT=on
      | [0
      | 0.018
      | 0.036
      | 0.054
      | 0.072
      | 0.09
      | 0.108
      | 0.126
      | 0.144
      | 0.162
      | 0.18
      | 0.198
      | 0.216
      | 0.234
      | 0.252
      | 0.27
      | 0.288
      | 0.306
      | 0.324
      | 0.342
      | 0.36
      | 0.378
      | 0.396
      | 0.414
      | 0.432
      | 0.45
      | 0.468
      | 0.486
      | 0.504
      | 0.522
      | 0.54
      | 0.558
      | 0.576
      | 0.594
      | 0.612
      | 0.63
      | 0.648
      | 0.666
      | 0.684
      | 0.702
      | 0.72
      | 0.738
      | 0.756
      | 0.774
      | 0.792
      | 0.81
      | 0.828
      | 0.846
      | 0.864
      | 0.882
      | 0.9
      | 0.918
      | 0.936
      | 0.954
      | 0.972
      | 0.99
      | 1.008
      | 1.026
      | 1.044
      | 1.062
      | 1.08
      | 1.098
      | 1.116
      | 1.134
      | 1.152
      | 1.17
      | 1.188
      | 1.206
      | 1.224
      | 1.242
      | 1.26
      | 1.278
      | 1.296
      | 1.314
      | 1.332
      | 1.35
      | 1.368
      | 1.386
      | 1.404
      | 1.422
      | 1.44
      | 1.458
      | 1.476
      | 1.494
      | 1.512
      | 1.53
      | 1.548
      | 1.566
      | 1.584
      | 1.602
      | 1.62
      | 1.638
      | 1.656
      | 1.674
      | 1.692
      | 1.71
      | 1.728
      | 1.746
      | 1.764
      | 1.782
      | 1.8
      | 1.818
      | 1.836
      | 1.854
      | 1.872
      | 1.89
      | 1.908
      | 1.926
      | 1.944
      | 1.962
      | 1.98
      | 1.998
      | 2.016
      | 2.034
      | 2.052
      | 2.07
      | 2.088
      | 2.106
      | 2.124
      | 2.142
      | 2.16
      | 2.178
      | 2.196
      | 2.214
      | 2.232
      | 2.25
      | 2.268
      | 2.286
      | 2.304
      | 2.322
      | 2.34
      | 2.358
      | 2.376
      | 2.394
      | 2.412
      | 2.43
      | 2.448
      | 2.466
      | 2.484
      | 2.502
      | 2.52
      | 2.538
      | 2.556
      | 2.574
      | 2.592
      | 2.61
      | 2.628
      | 2.646
      | 2.664
      | 2.682
      | 2.7
      | 2.718
      | 2.736
      | 2.754
      | 2.772
      | 2.79
      | 2.808
      | 2.826
      | 2.844
      | 2.862
      | 2.88
      | 2.898
      | 2.916
      | 2.934
      | 2.952
      | 2.97
      | 2.988
      | 3.006
      | 3.024
      | 3.042
      | 3.06
      | 3.078
      | 3.096
      | 3.114
      | 3.132
      | 3.15
      | 3.168
      | 3.186
      | 3.204
      | 3.222
      | 3.24
      | 3.258
      | 3.276
      | 3.294
      | 3.312
      | 3.33
      | 3.348
      | 3.366
      | 3.384
      | 3.402
      | 3.42
      | 3.438
      | 3.456
      | 3.474
      | 3.492
      | 3.51
      | 3.528
      | 3.546
      | 3.564
      | 3.582
      | 3.6
      | 3.61439994
      | 3.62879988
      | 3.64319982
      | 3.65759976
      | 3.6719997
      | 3.68639964
      | 3.70079958
      | 3.71519952
      | 3.72959946
      | 3.7439994
      | 3.75839934
      | 3.77279928
      | 3.78719922
      | 3.80159916
      | 3.8159991
      | 3.83039904
      | 3.84479898
      | 3.85919892
      | 3.87359886
      | 3.8879988
      | 3.90239874
      | 3.91679868
      | 3.93119862
      | 3.94559856
      | 3.9599985
      | 3.97439844
      | 3.98879838
      | 4.00319832
      | 4.01759826
      | 4.0319982
      | 4.04639814
      | 4.06079808
      | 4.07519802
      | 4.08959796
      | 4.1039979
      | 4.11839784
      | 4.13279778
      | 4.14719772
      | 4.16159766
      | 4.1759976
      | 4.19039754
      | 4.20479748
      | 4.21919742
      | 4.23359736
      | 4.2479973
      | 4.26239724
      | 4.27679718
      | 4.29119712
      | 4.30559706
      | 4.319997
      | 4.33439694
      | 4.34879688
      | 4.36319682
      | 4.37759676
      | 4.3919967
      | 4.40639664
      | 4.42079658
      | 4.43519652
      | 4.44959646
      | 4.4639964
      | 4.47839634
      | 4.49279628
      | 4.50719622
      | 4.52159616
      | 4.5359961
      | 4.55039604
      | 4.56479598
      | 4.57919592
      | 4.59359586
      | 4.6079958
      | 4.62239574
      | 4.63679568
      | 4.65119562
      | 4.66559556
      | 4.6799955
      | 4.69439544
      | 4.70879538
      | 4.72319532
      | 4.73759526
      | 4.7519952
      | 4.76639514
      | 4.78079508
      | 4.79519502
      | 4.80959496
      | 4.8239949
      | 4.83839484
      | 4.85279478
      | 4.86719472
      | 4.88159466
      | 4.8959946
      | 4.91039454
      | 4.92479448
      | 4.93919442
      | 4.95359436
      | 4.9679943
      | 4.98239424
      | 4.99679418
      | 5.01119412
      | 5.02559406
      | 5.039994
      | 5.05439394
      | 5.06879388
      | 5.08319382
      | 5.09759376
      | 5.1119937
      | 5.12639364
      | 5.14079358
      | 5.15519352
      | 5.16959346
      | 5.1839934
      | 5.19839334
      | 5.21279328
      | 5.22719322
      | 5.24159316
      | 5.2559931
      | 5.27039304
      | 5.28479298
      | 5.29919292
      | 5.31359286
      | 5.3279928
      | 5.34239274
      | 5.35679268
      | 5.37119262
      | 5.38559256
      | 5.3999925
      | 5.41439244
      | 5.42879238
      | 5.44319232
      | 5.45759226
      | 5.4719922
      | 5.48639214
      | 5.50079208
      | 5.51519202
      | 5.52959196
      | 5.5439919
      | 5.55839184
      | 5.57279178
      | 5.58719172
      | 5.60159166
      | 5.6159916
      | 5.63039154
      | 5.64479148
      | 5.65919142
      | 5.67359136
      | 5.6879913
      | 5.70239124
      | 5.71679118
      | 5.73119112
      | 5.74559106
      | 5.759991
      | 5.77439094
      | 5.78879088
      | 5.80319082
      | 5.81759076
      | 5.8319907
      | 5.84639064
      | 5.86079058
      | 5.87519052
      | 5.88959046
      | 5.9039904
      | 5.91839034
      | 5.93279028
      | 5.94719022
      | 5.96159016
      | 5.9759901
      | 5.99039004
      | 6.00478998
      | 6.01918992
      | 6.03358986
      | 6.0479898
      | 6.06238974
      | 6.07678968
      | 6.09118962
      | 6.10558956
      | 6.1199895
      | 6.13438944
      | 6.14878938
      | 6.16318932
      | 6.17758926
      | 6.1919892
      | 6.20638914
      | 6.22078908
      | 6.23518902
      | 6.24958896
      | 6.2639889
      | 6.27838884
      | 6.29278878
      | 6.30718872
      | 6.32158866
      | 6.3359886
      | 6.35038854
      | 6.36478848
      | 6.37918842
      | 6.39358836
      | 6.4079883
      | 6.42238824
      | 6.43678818
      | 6.45118812
      | 6.46558806
      | 6.479988
      | 6.49438794
      | 6.50878788
      | 6.52318782
      | 6.53758776
      | 6.5519877
      | 6.56638764
      | 6.58078758
      | 6.59518752
      | 6.60958746
      | 6.6239874
      | 6.63838734
      | 6.65278728
      | 6.66718722
      | 6.68158716
      | 6.6959871
      | 6.71038704
      | 6.72478698
      | 6.73918692
      | 6.75358686
      | 6.7679868
      | 6.78238674
      | 6.79678668
      | 6.81118662
      | 6.82558656
      | 6.8399865
      | 6.85438644
      | 6.86878638
      | 6.88318632
      | 6.89758626
      | 6.9119862
      | 6.92638614
      | 6.94078608
      | 6.95518602
      | 6.96958596
      | 6.9839859
      | 6.99838584
      | 7.01278578
      | 7.02718572
      | 7.04158566
      | 7.0559856
      | 7.07038554
      | 7.08478548
      | 7.09918542
      | 7.11358536
      | 7.1279853
      | 7.14238524
      | 7.15678518
      | 7.17118512
      | 7.18558506
      | 7.199985
      | 7.21438494
      | 7.22878488
      | 7.24318482
      | 7.25758476
      | 7.2719847
      | 7.28638464
      | 7.30078458
      | 7.31518452
      | 7.32958446
      | 7.3439844
      | 7.35838434
      | 7.37278428
      | 7.38718422
      | 7.40158416
      | 7.4159841
      | 7.43038404
      | 7.44478398
      | 7.45918392
      | 7.47358386
      | 7.4879838
      | 7.50238374
      | 7.51678368
      | 7.53118362
      | 7.54558356
      | 7.5599835
      | 7.57438344
      | 7.58878338
      | 7.60318332
      | 7.61758326
      | 7.6319832
      | 7.64638314
      | 7.66078308
      | 7.67518302
      | 7.68958296
      | 7.7039829
      | 7.71838284
      | 7.73278278
      | 7.74718272
      | 7.76158266
      | 7.7759826
      | 7.79038254
      | 7.80478248
      | 7.81918242
      | 7.83358236
      | 7.8479823
      | 7.86238224
      | 7.87678218
      | 7.89118212
      | 7.90558206
      | 7.919982
      | 7.93438194
      | 7.94878188
      | 7.96318182
      | 7.97758176
      | 7.9919817
      | 8.00638164
      | 8.02078158
      | 8.03518152
      | 8.04958146
      | 8.0639814
      | 8.07838134
      | 8.09278128
      | 8.10718122
      | 8.12158116
      | 8.123874581
      | 8.141874581
      | 8.159874581
      | 8.177874581
      | 8.195874581
      | 8.213874581
      | 8.231874581
      | 8.249874581
      | 8.267874581
      | 8.285874581
      | 8.303874581
      | 8.321874581
      | 8.339874581
      | 8.357874581
      | 8.375874581
      | 8.393874581
      | 8.411874581
      | 8.429874581
      | 8.447874581
      | 8.465874581
      | 8.483874581
      | 8.501874581
      | 8.519874581
      | 8.537874581
      | 8.555874581
      | 8.573874581
      | 8.591874581
      | 8.609874581
      | 8.627874581
      | 8.645874581
      | 8.663874581
      | 8.681874581
      | 8.699874581
      | 8.717874581
      | 8.735874581
      | 8.753874581
      | 8.771874581
      | 8.789874581
      | 8.807874581
      | 8.825874581
      | 8.843874581
      | 8.861874581
      | 8.879874581
      | 8.897874581
      | 8.915874581
      | 8.933874581
      | 8.951874581
      | 8.969874581
      | 8.987874581
      | 9.005874581
      | 9.023874581
      | 9.041874581
      | 9.059874581
      | 9.077874581
      | 9.095874581
      | 9.113874581
      | 9.131874581
      | 9.149874581
      | 9.167874581
      | 9.185874581
      | 9.203874581
      | 9.221874581
      | 9.239874581
      | 9.257874581
      | 9.275874581
      | 9.293874581
      | 9.311874581
      | 9.329874581
      | 9.347874581
      | 9.365874581
      | 9.383874581
      | 9.401874581
      | 9.419874581
      | 9.437874581
      | 9.455874581
      | 9.473874581
      | 9.491874581
      | 9.509874581
      | 9.527874581
      | 9.545874581
      | 9.563874581
      | 9.581874581
      | 9.599874581
      | 9.617874581
      | 9.635874581
      | 9.653874581
      | 9.671874581
      | 9.689874581
      | 9.707874581
      | 9.725874581
      | 9.743874581
      | 9.761874581
      | 9.779874581
      | 9.797874581
      | 9.815874581
      | 9.833874581
      | 9.851874581
      | 9.869874581
      | 9.887874581
      | 9.905874581
      | 9.923874581
      | 9.941874581
      | 9.959874581
      | 9.977874581
      | 9.995874581
      | 10.01387458
      | 10.03187458
      | 10.04987458
      | 10.06787458
      | 10.08587458
      | 10.10387458
      | 10.12187458
      | 10.13987458
      | 10.15787458
      | 10.17587458
      | 10.19387458
      | 10.21187458
      | 10.22987458
      | 10.24787458
      | 10.26587458
      | 10.28387458
      | 10.30187458
      | 10.31987458
      | 10.33787458
      | 10.35587458
      | 10.37387458
      | 10.39187458
      | 10.40987458
      | 10.42787458
      | 10.44587458
      | 10.46387458
      | 10.48187458
      | 10.49987458
      | 10.51787458
      | 10.53587458
      | 10.55387458
      | 10.57187458
      | 10.58987458
      | 10.60787458
      | 10.62587458
      | 10.64387458
      | 10.66187458
      | 10.67987458
      | 10.69787458
      | 10.71587458
      | 10.73387458
      | 10.75187458
      | 10.76987458
      | 10.78787458
      | 10.80587458
      | 10.82387458
      | 10.84187458
      | 10.85987458
      | 10.87787458
      | 10.89587458
      | 10.91387458
      | 10.93187458
      | 10.94987458
      | 10.96787458
      | 10.98587458
      | 11.00387458
      | 11.02187458
      | 11.03987458
      | 11.05787458
      | 11.07587458
      | 11.09387458
      | 11.11187458
      | 11.12987458
      | 11.14787458
      | 11.16587458
      | 11.18387458
      | 11.20187458
      | 11.21987458
      | 11.23787458
      | 11.25587458
      | 11.27387458
      | 11.29187458
      | 11.30987458
      | 11.32787458
      | 11.34587458
      | 11.36387458
      | 11.38187458
      | 11.39987458
      | 11.41787458
      | 11.43587458
      | 11.45387458
      | 11.47187458
      | 11.48987458
      | 11.50787458
      | 11.52587458
      | 11.54387458
      | 11.56187458
      | 11.57987458
      | 11.59787458
      | 11.61587458
      | 11.63387458
      | 11.65187458
      | 11.66987458
      | 11.68787458
      | 11.70587458
      | 11.72387458
      | ]*4/3
      | [0
      | 0
      | 0
      | 0
      | 0
      | 0
      | 0
      | 0
      | 0
      | 0
      | 0
      | 0
      | 0
      | 0
      | 0
      | 0
      | 0
      | 0
      | 0
      | 0
      | 0
      | 0
      | 0
      | 0
      | 0
      | 0
      | 0
      | 0
      | 0
      | 0
      | 0
      | 0
      | 0
      | 0
      | 0
      | 0
      | 0
      | 0
      | 0
      | 0
      | 0
      | 0
      | 0
      | 0
      | 0
      | 0
      | 0
      | 0
      | 0
      | 0
      | 0
      | 0
      | 0
      | 0
      | 0
      | 0
      | 0
      | 0
      | 0
      | 0
      | 0
      | 0
      | 0
      | 0
      | 0
      | 0
      | 0
      | 0
      | 0
      | 0
      | 0
      | 0
      | 0
      | 0
      | 0
      | 0
      | 0
      | 0
      | 0
      | 0
      | 0
      | 0
      | 0
      | 0
      | 0
      | 0
      | 0
      | 0
      | 0
      | 0
      | 0
      | 0
      | 0
      | 0
      | 0
      | 0
      | 0
      | 0
      | 0
      | 0
      | 0
      | 0
      | 0
      | 0
      | 0
      | 0
      | 0
      | 0
      | 0
      | 0
      | 0
      | 0
      | 0
      | 0
      | 0
      | 0
      | 0
      | 0
      | 0
      | 0
      | 0
      | 0
      | 0
      | 0
      | 0
      | 0
      | 0
      | 0
      | 0
      | 0
      | 0
      | 0
      | 0
      | 0
      | 0
      | 0
      | 0
      | 0
      | 0
      | 0
      | 0
      | 0
      | 0
      | 0
      | 0
      | 0
      | 0
      | 0
      | 0
      | 0
      | 0
      | 0
      | 0
      | 0
      | 0
      | 0
      | 0
      | 0
      | 0
      | 0
      | 0
      | 0
      | 0
      | 0
      | 0
      | 0
      | 0
      | 0
      | 0
      | 0
      | 0
      | 0
      | 0
      | 0
      | 0
      | 0
      | 0
      | 0
      | 0
      | 0
      | 0
      | 0
      | 0
      | 0
      | 0
      | 0
      | 0
      | 0
      | 0
      | 0
      | 0
      | 0
      | 0
      | 0
      | 0
      | 0
      | 0
      | 0
      | 0
      | 0
      | 0.286478902
      | 0.859436707
      | 1.432394512
      | 2.005352317
      | 2.578310122
      | 3.151267927
      | 3.724225732
      | 4.297183537
      | 4.870141342
      | 5.443099147
      | 6.016056951
      | 6.589014756
      | 7.161972561
      | 7.734930366
      | 8.307888171
      | 8.880845976
      | 9.453803781
      | 10.02676159
      | 10.59971939
      | 11.1726772
      | 11.745635
      | 12.31859281
      | 12.89155061
      | 13.46450842
      | 14.03746622
      | 14.61042403
      | 15.18338183
      | 15.75633963
      | 16.32929744
      | 16.90225524
      | 17.47521305
      | 18.04817085
      | 18.62112866
      | 19.19408646
      | 19.76704427
      | 20.34000207
      | 20.91295988
      | 21.48591768
      | 22.05887549
      | 22.63183329
      | 23.2047911
      | 23.7777489
      | 24.35070671
      | 24.92366451
      | 25.49662232
      | 26.06958012
      | 26.64253793
      | 27.21549573
      | 27.78845354
      | 28.36141134
      | 28.93436915
      | 29.50732695
      | 30.08028476
      | 30.65324256
      | 31.22620037
      | 31.79915817
      | 32.37211598
      | 32.94507378
      | 33.51803159
      | 34.09098939
      | 34.6639472
      | 35.236905
      | 35.80986281
      | 36.38282061
      | 36.95577842
      | 37.52873622
      | 38.10169403
      | 38.67465183
      | 39.24760964
      | 39.82056744
      | 40.39352525
      | 40.96648305
      | 41.53944086
      | 42.11239866
      | 42.68535647
      | 43.25831427
      | 43.83127208
      | 44.40422988
      | 44.97718768
      | 45.55014549
      | 46.12310329
      | 46.6960611
      | 47.2690189
      | 47.84197671
      | 48.41493451
      | 48.98789232
      | 49.56085012
      | 50.13380793
      | 50.70676573
      | 51.27972354
      | 51.85268134
      | 52.42563915
      | 52.99859695
      | 53.57155476
      | 54.14451256
      | 54.71747037
      | 55.29042817
      | 55.86338598
      | 56.43634378
      | 57.00930159
      | 57.58225939
      | 58.1552172
      | 58.728175
      | 59.30113281
      | 59.87409061
      | 60.44704842
      | 61.02000622
      | 61.59296403
      | 62.16592183
      | 62.73887964
      | 63.31183744
      | 63.88479525
      | 64.45775305
      | 65.03071086
      | 65.60366866
      | 66.17662647
      | 66.74958427
      | 67.32254208
      | 67.89549988
      | 68.46845769
      | 69.04141549
      | 69.6143733
      | 70.1873311
      | 70.76028891
      | 71.33324671
      | 71.90620452
      | 72.47916232
      | 73.05212013
      | 73.62507793
      | 74.19803574
      | 74.77099354
      | 75.34395134
      | 75.91690915
      | 76.48986695
      | 77.06282476
      | 77.63578256
      | 78.20874037
      | 78.78169817
      | 79.35465598
      | 79.92761378
      | 80.50057159
      | 81.07352939
      | 81.6464872
      | 82.219445
      | 82.79240281
      | 83.36536061
      | 83.93831842
      | 84.51127622
      | 85.08423403
      | 85.65719183
      | 86.23014964
      | 86.80310744
      | 87.37606525
      | 87.94902305
      | 88.52198086
      | 89.09493866
      | 89.66789647
      | 90.24085427
      | 90.81381208
      | 91.38676988
      | 91.95972769
      | 92.53268549
      | 93.1056433
      | 93.6786011
      | 94.25155891
      | 94.82451671
      | 95.39747452
      | 95.97043232
      | 96.54339013
      | 97.11634793
      | 97.68930574
      | 98.26226354
      | 98.83522135
      | 99.40817915
      | 99.98113696
      | 100.5540948
      | 101.1270526
      | 101.7000104
      | 102.2729682
      | 102.845926
      | 103.4188838
      | 103.9918416
      | 104.5647994
      | 105.1377572
      | 105.710715
      | 106.2836728
      | 106.8566306
      | 107.4295884
      | 108.0025462
      | 108.575504
      | 109.1484618
      | 109.7214196
      | 110.2943774
      | 110.8673352
      | 111.4402931
      | 112.0132509
      | 112.5862087
      | 113.1591665
      | 113.7321243
      | 114.3050821
      | 114.8780399
      | 115.4509977
      | 116.0239555
      | 116.5969133
      | 117.1698711
      | 117.7428289
      | 118.3157867
      | 118.8887445
      | 119.4617023
      | 120.0346601
      | 120.6076179
      | 121.1805757
      | 121.7535335
      | 122.3264913
      | 122.8994492
      | 123.472407
      | 124.0453648
      | 124.6183226
      | 125.1912804
      | 125.7642382
      | 126.337196
      | 126.9101538
      | 127.4831116
      | 128.0560694
      | 128.6290272
      | 129.201985
      | 129.7749428
      | 130.3479006
      | 130.9208584
      | 131.4938162
      | 132.066774
      | 132.6397318
      | 133.2126896
      | 133.7856474
      | 134.3586053
      | 134.9315631
      | 135.5045209
      | 136.0774787
      | 136.6504365
      | 137.2233943
      | 137.7963521
      | 138.3693099
      | 138.9422677
      | 139.5152255
      | 140.0881833
      | 140.6611411
      | 141.2340989
      | 141.8070567
      | 142.3800145
      | 142.9529723
      | 143.5259301
      | 144.0988879
      | 144.6718457
      | 145.2448035
      | 145.8177613
      | 146.3907192
      | 146.963677
      | 147.5366348
      | 148.1095926
      | 148.6825504
      | 149.2555082
      | 149.828466
      | 150.4014238
      | 150.9743816
      | 151.5473394
      | 152.1202972
      | 152.693255
      | 153.2662128
      | 153.8391706
      | 154.4121284
      | 154.9850862
      | 155.558044
      | 156.1310018
      | 156.7039596
      | 157.2769174
      | 157.8498753
      | 158.4228331
      | 158.9957909
      | 159.5687487
      | 160.1417065
      | 160.7146643
      | 161.2876221
      | 161.8605799
      | 162.4335377
      | 163.0064955
      | 163.5794533
      | 164.1524111
      | 164.7253689
      | 165.2983267
      | 165.8712845
      | 166.4442423
      | 167.0172001
      | 167.5901579
      | 168.1631157
      | 168.7360735
      | 169.3090313
      | 169.8819892
      | 170.454947
      | 171.0279048
      | 171.6008626
      | 172.1738204
      | 172.7467782
      | 173.319736
      | 173.8926938
      | 174.4656516
      | 175.0386094
      | 175.6115672
      | 176.184525
      | 176.7574828
      | 177.3304406
      | 177.9033984
      | 178.4763562
      | 179.049314
      | 179.6222718
      | 179.9543769
      | 180.0000031
      | 180.0000031
      | 180.0000031
      | 180.0000031
      | 180.0000031
      | 180.0000031
      | 180.0000031
      | 180.0000031
      | 180.0000031
      | 180.0000031
      | 180.0000031
      | 180.0000031
      | 180.0000031
      | 180.0000031
      | 180.0000031
      | 180.0000031
      | 180.0000031
      | 180.0000031
      | 180.0000031
      | 180.0000031
      | 180.0000031
      | 180.0000031
      | 180.0000031
      | 180.0000031
      | 180.0000031
      | 180.0000031
      | 180.0000031
      | 180.0000031
      | 180.0000031
      | 180.0000031
      | 180.0000031
      | 180.0000031
      | 180.0000031
      | 180.0000031
      | 180.0000031
      | 180.0000031
      | 180.0000031
      | 180.0000031
      | 180.0000031
      | 180.0000031
      | 180.0000031
      | 180.0000031
      | 180.0000031
      | 180.0000031
      | 180.0000031
      | 180.0000031
      | 180.0000031
      | 180.0000031
      | 180.0000031
      | 180.0000031
      | 180.0000031
      | 180.0000031
      | 180.0000031
      | 180.0000031
      | 180.0000031
      | 180.0000031
      | 180.0000031
      | 180.0000031
      | 180.0000031
      | 180.0000031
      | 180.0000031
      | 180.0000031
      | 180.0000031
      | 180.0000031
      | 180.0000031
      | 180.0000031
      | 180.0000031
      | 180.0000031
      | 180.0000031
      | 180.0000031
      | 180.0000031
      | 180.0000031
      | 180.0000031
      | 180.0000031
      | 180.0000031
      | 180.0000031
      | 180.0000031
      | 180.0000031
      | 180.0000031
      | 180.0000031
      | 180.0000031
      | 180.0000031
      | 180.0000031
      | 180.0000031
      | 180.0000031
      | 180.0000031
      | 180.0000031
      | 180.0000031
      | 180.0000031
      | 180.0000031
      | 180.0000031
      | 180.0000031
      | 180.0000031
      | 180.0000031
      | 180.0000031
      | 180.0000031
      | 180.0000031
      | 180.0000031
      | 180.0000031
      | 180.0000031
      | 180.0000031
      | 180.0000031
      | 180.0000031
      | 180.0000031
      | 180.0000031
      | 180.0000031
      | 180.0000031
      | 180.0000031
      | 180.0000031
      | 180.0000031
      | 180.0000031
      | 180.0000031
      | 180.0000031
      | 180.0000031
      | 180.0000031
      | 180.0000031
      | 180.0000031
      | 180.0000031
      | 180.0000031
      | 180.0000031
      | 180.0000031
      | 180.0000031
      | 180.0000031
      | 180.0000031
      | 180.0000031
      | 180.0000031
      | 180.0000031
      | 180.0000031
      | 180.0000031
      | 180.0000031
      | 180.0000031
      | 180.0000031
      | 180.0000031
      | 180.0000031
      | 180.0000031
      | 180.0000031
      | 180.0000031
      | 180.0000031
      | 180.0000031
      | 180.0000031
      | 180.0000031
      | 180.0000031
      | 180.0000031
      | 180.0000031
      | 180.0000031
      | 180.0000031
      | 180.0000031
      | 180.0000031
      | 180.0000031
      | 180.0000031
      | 180.0000031
      | 180.0000031
      | 180.0000031
      | 180.0000031
      | 180.0000031
      | 180.0000031
      | 180.0000031
      | 180.0000031
      | 180.0000031
      | 180.0000031
      | 180.0000031
      | 180.0000031
      | 180.0000031
      | 180.0000031
      | 180.0000031
      | 180.0000031
      | 180.0000031
      | 180.0000031
      | 180.0000031
      | 180.0000031
      | 180.0000031
      | 180.0000031
      | 180.0000031
      | 180.0000031
      | 180.0000031
      | 180.0000031
      | 180.0000031
      | 180.0000031
      | 180.0000031
      | 180.0000031
      | 180.0000031
      | 180.0000031
      | 180.0000031
      | 180.0000031
      | 180.0000031
      | 180.0000031
      | 180.0000031
      | 180.0000031
      | 180.0000031
      | 180.0000031
      | 180.0000031
      | 180.0000031
      | 180.0000031
      | 180.0000031
      | 180.0000031
      | 180.0000031
      | 180.0000031
      | 180.0000031
      | 180.0000031
      | 180.0000031
      | 180
      | ]
  15epoch : Subsystem  mask{pi_input_1_delayed_1=[0;0;0;0], pi_input_1_delayed_2=[0;0;0;0], pi_input_1_delayed_3=[0;0;0;0]}
      mask prompts: pi_input_1_delayed_1 "Preprocessed initial input 1 state at timestep 0."; pi_input_1_delayed_2 "Preprocessed initial input 1 state at timestep -1."; pi_input_1_delayed_3 "Preprocessed initial input 1 state at timestep -2."
      mask help: Time Delay Neural Network
      mask Display: e = 0.06;c1 = [120 150 230]/255;c2 = ([120 150 230]+0)/383;c3 = ([120 150 230]+128)/383;patch([0 1 1 0],[0 0 1 1],c1);patch([0 1 1 1-e 1-e 0+e],[0 0 1 1-e 0+e 0+e],c2);patch([0 0 1 1-e 0+e 0+e],[0 1 1 1-e 1-e 0+e],c3);plot([0 1 1 0 0],[0 0 1 1 0]);fprintf('NNET');port_label('input',1,' x');port_label('output',1,'y ');
  15epoch_2 用的0.2s_0.02_2的数据 : Subsystem  mask{pi_input_1_delayed_1=[0;0;0;0], pi_input_1_delayed_2=[0;0;0;0], pi_input_1_delayed_3=[0;0;0;0]}
      mask prompts: pi_input_1_delayed_1 "Preprocessed initial input 1 state at timestep 0."; pi_input_1_delayed_2 "Preprocessed initial input 1 state at timestep -1."; pi_input_1_delayed_3 "Preprocessed initial input 1 state at timestep -2."
      mask help: Time Delay Neural Network
      mask Display: e = 0.06;c1 = [120 150 230]/255;c2 = ([120 150 230]+0)/383;c3 = ([120 150 230]+128)/383;patch([0 1 1 0],[0 0 1 1],c1);patch([0 1 1 1-e 1-e 0+e],[0 0 1 1-e 0+e 0+e],c2);patch([0 0 1 1-e 0+e 0+e],[0 1 1 1-e 1-e 0+e],c3);plot([0 1 1 0 0],[0 0 1 1 0]);fprintf('NNET');port_label('input',1,' x');port_label('output',1,'y ');
  60:360训练的 : Subsystem  mask{pi_input_1_delayed_1=[0;0;0;0], pi_input_1_delayed_2=[0;0;0;0], pi_input_1_delayed_3=[0;0;0;0]}
      mask prompts: pi_input_1_delayed_1 "Preprocessed initial input 1 state at timestep 0."; pi_input_1_delayed_2 "Preprocessed initial input 1 state at timestep -1."; pi_input_1_delayed_3 "Preprocessed initial input 1 state at timestep -2."
      mask help: Time Delay Neural Network
      mask Display: e = 0.06;c1 = [120 150 230]/255;c2 = ([120 150 230]+0)/383;c3 = ([120 150 230]+128)/383;patch([0 1 1 0],[0 0 1 1],c1);patch([0 1 1 1-e 1-e 0+e],[0 0 1 1-e 0+e 0+e],c2);patch([0 0 1 1-e 0+e 0+e],[0 1 1 1-e 1-e 0+e],c3);plot([0 1 1 0 0],[0 0 1 1 0]);fprintf('NNET');port_label('input',1,' x');port_label('output',1,'y ');
  Abs : Abs
  Add : Sum  Inputs=+-
  Add1 : Sum  Inputs=+-
  CarSim S-Function : Solver_SF/CarSim S-Function  Priority=1  VehicleCode=i_i  SIMFILE=simfile.sim
  Clock1 : Clock
  Clock2 : Clock
  Constant2 : Constant  Value=0
  Demux : Demux  Outputs=9
  Demux1 : Demux  Outputs=2
  Gain : Gain  Gain=3.6
  Gain1 : Gain  Gain=1/3.6
  Gain10 : Gain  Gain=0.8
  Gain11 : Gain  Gain=1/0.02
  Gain2 : Gain  Gain=3.14/180
  Gain3 : Gain  Gain=0.6/0.8
  Gain4 : Gain  Gain=1/0.01
  Gain5 : Gain  Gain=180/3.14
  Gain6 : Gain  Gain=16.28
  Gain7 : Gain
  Mux1 : Mux  Inputs=3
  Mux3 : Mux  Inputs=6
  Mux4 : Mux  Inputs=2
  Mux5 : Mux  Inputs=3
  "PID " : simulink/Continuous/PID Controller  Controller=PID  TimeDomain=Discrete-time  SampleTime=0.01  IntegratorMethod=Forward Euler  FilterMethod=Forward Euler  Form=Parallel  UseFilter=off  ControllerParametersSource=internal  P=1  I=0  D=-0.01  N=10  InitialConditionSource=internal  InitialConditionForIntegrator=0  InitialConditionForFilter=0  ExternalReset=none  LimitOutput=off  UpperSaturationLimit=inf  LowerSaturationLimit=-inf  LinearizeAsGain=off  AntiWindupMode=none  Kb=1  TrackingMode=off  Kt=1  PParamMin=[]  PParamMax=[]  IParamMin=[]  IParamMax=[]  DParamMin=[]  DParamMax=[]  NParamMin=[]  NParamMax=[]  KbParamMin=[]  KbParamMax=[]  KtParamMin=[]  KtParamMax=[]  POutMin=[]  POutMax=[]  IOutMin=[]  IOutMax=[]  DOutMin=[]  DOutMax=[]  NOutMin=[]  NOutMax=[]  KbOutMin=[]  KbOutMax=[]  KtOutMin=[]  KtOutMax=[]  IntegratorOutMin=[]  IntegratorOutMax=[]  FilterOutMin=[]  FilterOutMax=[]  SumOutMin=[]  SumOutMax=[]  SumI1OutMin=[]  SumI1OutMax=[]  SumI2OutMin=[]  SumI2OutMax=[]  SumI3OutMin=[]  SumI3OutMax=[]  SumDOutMin=[]  SumDOutMax=[]  SaturationOutMin=[]  SaturationOutMax=[]  IntegratorContinuousStateAttributes=''  IntegratorStateMustResolveToSignalObject=off  IntegratorRTWStateStorageClass=Auto  FilterContinuousStateAttributes=''  FilterStateMustResolveToSignalObject=off  FilterRTWStateStorageClass=Auto  DifferentiatorICPrevScaledInput=0  DifferentiatorOutMin=[]  DifferentiatorOutMax=[]
  PID 1 : simulink/Continuous/PID Controller  Controller=PID  TimeDomain=Discrete-time  SampleTime=0.01  IntegratorMethod=Forward Euler  FilterMethod=Forward Euler  Form=Parallel  UseFilter=off  ControllerParametersSource=internal  P=1  I=-2  D=0  N=10  InitialConditionSource=internal  InitialConditionForIntegrator=0  InitialConditionForFilter=0  ExternalReset=either  LimitOutput=off  UpperSaturationLimit=inf  LowerSaturationLimit=-inf  LinearizeAsGain=off  AntiWindupMode=none  Kb=1  TrackingMode=off  Kt=1  PParamMin=[]  PParamMax=[]  IParamMin=[]  IParamMax=[]  DParamMin=[]  DParamMax=[]  NParamMin=[]  NParamMax=[]  KbParamMin=[]  KbParamMax=[]  KtParamMin=[]  KtParamMax=[]  POutMin=[]  POutMax=[]  IOutMin=[]  IOutMax=[]  DOutMin=[]  DOutMax=[]  NOutMin=[]  NOutMax=[]  KbOutMin=[]  KbOutMax=[]  KtOutMin=[]  KtOutMax=[]  IntegratorOutMin=[]  IntegratorOutMax=[]  FilterOutMin=[]  FilterOutMax=[]  SumOutMin=[]  SumOutMax=[]  SumI1OutMin=[]  SumI1OutMax=[]  SumI2OutMin=[]  SumI2OutMax=[]  SumI3OutMin=[]  SumI3OutMax=[]  SumDOutMin=[]  SumDOutMax=[]  SaturationOutMin=[]  SaturationOutMax=[]  IntegratorContinuousStateAttributes=''  IntegratorStateMustResolveToSignalObject=off  IntegratorRTWStateStorageClass=Auto  FilterContinuousStateAttributes=''  FilterStateMustResolveToSignalObject=off  FilterRTWStateStorageClass=Auto  DifferentiatorICPrevScaledInput=0  DifferentiatorOutMin=[]  DifferentiatorOutMax=[]
  PID弯道 : Scope  NumInputPorts=2
  PID直道 : Scope  NumInputPorts=2
  Random Number : RandomNumber  Variance=0.0005  SampleTime=0.1
  S-Function : S-Function  FunctionName=MY_MPCController3_180  SFunctionDeploymentMode=off  EnableBusSupport=off
  Saturation1 : Saturate  UpperLimit=0.08  LowerLimit=-0.08
  Subtract{1,7..9} (4 alike) : Sum  Inputs=+-
  Subtract11 : Sum
  Subtract2 : Sum
  Subtract3 : Sum
  Switch1 : Switch  Criteria=u2 > Threshold  Threshold=1
  Switch3 : Switch  Criteria=u2 > Threshold  Threshold=2.5
  To Workspace : ToWorkspace  VariableName=x_real  SaveFormat=Timeseries  SampleTime=-1
  To Workspace1 : ToWorkspace  VariableName=y_real  SaveFormat=Timeseries  SampleTime=-1
  To Workspace2 : ToWorkspace  VariableName=x_predict  SaveFormat=Timeseries  SampleTime=-1
  To Workspace3 : ToWorkspace  VariableName=y_predict  SaveFormat=Timeseries  SampleTime=-1
  To Workspace4 : ToWorkspace  VariableName=v_predict  SaveFormat=Timeseries  SampleTime=-1
  To Workspace5 : ToWorkspace  VariableName=v_real  SaveFormat=Timeseries  SampleTime=-1
  To Workspace6 : ToWorkspace  VariableName=steer_torque  SaveFormat=Timeseries  SampleTime=-1
  To Workspace7 : ToWorkspace  VariableName=Ay  SaveFormat=Timeseries  SampleTime=-1
  To Workspace8 : ToWorkspace  VariableName=Vy  SaveFormat=Timeseries  SampleTime=-1
  Unit Delay : UnitDelay  SampleTime=-1
  Unit Delay1 : UnitDelay  SampleTime=-1
  Unit Delay2 : UnitDelay  SampleTime=-1
  XY Graph : simulink/Sinks/XY Graph  xmin=0  xmax=50  ymin=-5  ymax=25  st=-1
  XY Graph1 : simulink/Sinks/XY Graph  xmin=0  xmax=50  ymin=-5  ymax=25  st=-1
  X误差 : Scope
  YAW偏差 : Scope
  Y误差 : Scope
  Zero-Order Hold{,1,7,12..13} (5 alike) : ZeroOrderHold  SampleTime=0.01
  Zero-Order Hold{2..6,8..11} (9 alike) : ZeroOrderHold  SampleTime=0.05
  omega : ToWorkspace  VariableName=omega  SaveFormat=Timeseries  SampleTime=-1
  real车速km/h : Scope
  yaw : Scope
  yaw变化率 : Scope
  仿真yaw : Scope
  前轮角度rad : Scope
  前轮角速度rad/s : Scope
  前轮转角 ° : Scope  NumInputPorts=2
  前轮转角 °1 : Scope  NumInputPorts=2
  前轮转角控制量rad : ToWorkspace  VariableName=delta_predict  SaveFormat=Timeseries  SampleTime=-1
  前轮转角控制量rad' : Scope
  前轮转角控制量rad1 : ToWorkspace  VariableName=delta_predict2  SaveFormat=Timeseries  SampleTime=-1
  实际前轮转角rad : ToWorkspace  VariableName=delta_real  SaveFormat=Timeseries  SampleTime=-1
  实际前轮转角rad' : Scope
  延迟时间 : Gain  Gain=0.2
  方向盘控制量 rad : Scope
  方向盘转矩 : Scope
  方向盘随机误差 rad : Scope
  横向加速度 : Scope
  横向速度 : Scope
  没有延时 °1 : Scope  NumInputPorts=2
  补偿 : Scope
  补偿后/实际值对比 : Scope  NumInputPorts=2
  补偿后/控制量 : Scope  NumInputPorts=2
  车速 : Constant  Value=15
  限制前/后 : Scope  NumInputPorts=2
  除去了predict-real重新训练 用的0.2s_0.02_2的数据 : Subsystem  mask{pi_input_1_delayed_1=[0;0;0], pi_input_1_delayed_2=[0;0;0], pi_input_1_delayed_3=[0;0;0]}
      mask prompts: pi_input_1_delayed_1 "Preprocessed initial input 1 state at timestep 0."; pi_input_1_delayed_2 "Preprocessed initial input 1 state at timestep -1."; pi_input_1_delayed_3 "Preprocessed initial input 1 state at timestep -2."
      mask help: Time Delay Neural Network
      mask Display: e = 0.06;c1 = [120 150 230]/255;c2 = ([120 150 230]+0)/383;c3 = ([120 150 230]+128)/383;patch([0 1 1 0],[0 0 1 1],c1);patch([0 1 1 1-e 1-e 0+e],[0 0 1 1-e 0+e 0+e],c2);patch([0 0 1 1-e 0+e 0+e],[0 1 1 1-e 1-e 0+e],c3);plot([0 1 1 0 0],[0 0 1 1 0]);fprintf('NNET');port_label('input',1,' x');port_label('output',1,'y ');
  wires:
  CarSim S-Function/1 -> Demux/1
  Demux/3 -> 仿真yaw/1, Subtract9/2, Mux1/3
  Demux/2 -> Zero-Order Hold8/1, Subtract8/2, XY Graph1/2, Mux1/2
  S-Function/1 -> Demux1/1
  Unit Delay/1 -> Mux3/1
  Demux1/1 -> Gain/1
  Demux1/2 -> Subtract3/2, 补偿后/实际值对比/1, 0.05s1/1, 前轮转角控制量rad'/1, 前轮转角控制量rad/1, 前轮转角 °1/1, Add/1, 0.05s2/1, 前轮角度rad/1, Mux5/1, Subtract1/1  "现在期望量"
  Zero-Order Hold/1 -> 1-D Lookup yaw/1, 1-D Lookup x/1, 1-D Lookup y/1
  1-D Lookup x/1 -> To Workspace2/1, XY Graph/1, Subtract7/1, Mux3/2  "x"
  1-D Lookup y/1 -> XY Graph/2, To Workspace3/1, Subtract8/1, Mux3/3  "y"
  Mux1/1 -> Unit Delay/1
  Clock1/1 -> Zero-Order Hold/1
  Mux3/1 -> S-Function/1
  1-D Lookup yaw/1 -> Subtract9/1, yaw/1, Add1/1, 0.05s3/1, Mux3/4  "yaw"
  Demux/1 -> Mux1/1, XY Graph1/1, Zero-Order Hold9/1, Subtract7/2
  Mux4/1 -> CarSim S-Function/1
  车速/1 -> To Workspace4/1, Gain1/1
  Demux/6 -> Zero-Order Hold3/1, 前轮转角 °/1  "1"
  Random Number/1 -> 方向盘随机误差 rad/1
  Subtract2/1 -> 方向盘控制量 rad/1, Gain5/1
  Gain6/1 -> Subtract2/1
  Demux/4 -> Unit Delay1/1, Zero-Order Hold2/1  "v(km/h)"
  Unit Delay1/1 -> real车速km/h/1, Mux3/5
  Demux/7 -> Zero-Order Hold1/1
  Zero-Order Hold1/1 -> Mux5/2, 方向盘转矩/1, To Workspace6/1
  Zero-Order Hold3/1 -> 前轮转角 °/2, Gain2/1  "2"
  Zero-Order Hold2/1 -> To Workspace5/1
  Mux5/1 -> 除去了predict-real重新训练 用的0.2s_0.02_2的数据/1(x)
  Gain2/1 -> 实际前轮转角rad'/1, Subtract11/1, Subtract1/2, 实际前轮转角rad/1  "实际前轮转角rad"
  Gain1/1 -> Mux3/6
  Subtract7/1 -> Zero-Order Hold4/1
  Subtract8/1 -> Zero-Order Hold5/1
  Zero-Order Hold4/1 -> X误差/1
  Zero-Order Hold5/1 -> Y误差/1
  Subtract9/1 -> Zero-Order Hold6/1
  Zero-Order Hold6/1 -> YAW偏差/1
  Gain/1 -> Mux4/1
  Gain11/1 -> 前轮角速度rad/s/1, Mux5/3, omega/1, 延迟时间/1  "前轮角速度rad/s"
  Zero-Order Hold12/1 -> 前轮转角 °1/2, Add/2
  Gain10/1 -> Gain11/1
  Add/1 -> Gain10/1
  0.15s/1 -> Subtract11/2  "0.3秒前控制+补偿"
  Subtract11/1 -> 补偿后/控制量/2
  Subtract3/1 -> Gain6/1, 没有延时 °1/2, Zero-Order Hold7/1, 0.2s1/1  "补偿后的控制量"
  Saturation1/1 -> Switch3/1, 限制前/后/2
  Clock2/1 -> Switch3/2
  Switch3/1 -> Subtract3/1
  Constant2/1 -> Switch3/3
  延迟时间/1 -> Gain7/1, Gain3/1, 补偿/1, 0.15s/1
  0.05s1/1 -> 补偿后/控制量/1
  0.2s1/1 -> 补偿后/实际值对比/2  "0.2s前补偿后的控制量"
  Zero-Order Hold7/1 -> 前轮转角控制量rad1/1, 没有延时 °1/1
  "PID "/1 -> Switch1/1, PID弯道/2  "弯道"
  0.05s3/1 -> Zero-Order Hold13/1
  Add1/1 -> Gain4/1
  Gain4/1 -> yaw变化率/1, Abs/1
  除去了predict-real重新训练 用的0.2s_0.02_2的数据/1(y) -> ?
  PID 1/1 -> PID直道/2, Unit Delay2/1, Switch1/3  "直道"
  Switch1/1 -> Saturation1/1, 限制前/后/1
  Gain7/1 -> PID弯道/1, "PID "/1
  Gain3/1 -> PID 1/1, PID直道/1
  Zero-Order Hold8/1 -> To Workspace1/1
  Zero-Order Hold9/1 -> To Workspace/1
  Demux/8 -> Zero-Order Hold10/1
  Zero-Order Hold10/1 -> 横向加速度/1, To Workspace7/1
  Demux/9 -> Zero-Order Hold11/1
  Zero-Order Hold11/1 -> 横向速度/1, To Workspace8/1
  0.05s2/1 -> Zero-Order Hold12/1
  Zero-Order Hold13/1 -> Add1/2
  Gain5/1 -> 0.2s/1
  0.2s/1 -> Mux4/2
  Abs/1 -> Switch1/2
  Unit Delay2/1 -> PID 1/2
